simulink model "RB_KAIROS_impControl_compensation"  (R2020b)
settings: Solver=ode4  StartTime=0.0  StopTime=t_end  FixedStep=Ts  RelTol=1e-3
values from neighbouring files (symbols this model uses):
  am = 0.3    [RB_KAIROS_ImpControl_OpSpace_quat_2020b_safety_main.m]
  am_r = 0.3    [RB_KAIROS_ImpControl_OpSpace_quat_2020b_safety_main.m]
  Kc = diag(50*ones(6,1))    [RB_KAIROS_ImpControl_OpSpace_quat_2020b_safety_main.m]
  Kp = 2*[400;400;400;400;0;0;0]    [RB_KAIROS_ImpControl_OpSpace_quat_2020b_safety_main.m]
  Kv = [1000;1000;1000;[300;300;300;300;300;300;300]]    [RB_KAIROS_ImpControl_OpSpace_quat_2020b_safety_main.m]
  model_sample_time = 0.001    [RB_KAIROS_ImpControl_OpSpace_quat_2020b_safety_main.m]
  q_dot_0 = zeros(10,1)    [RB_KAIROS_ImpControl_OpSpace_quat_2020b_safety_main.m]
  T_i = K    [RB_KAIROS_ImpControl_OpSpace_quat_2020b_safety_main.m]
  tau_ext = [0 0 0 0 0 0 0 0 0 0 0]    [RB_KAIROS_ImpControl_OpSpace_quat_2020b_safety_main.m]
  v_SMU = 10    [RB_KAIROS_ImpControl_OpSpace_quat_2020b_safety_main.m]
  vm = 0.5    [RB_KAIROS_ImpControl_OpSpace_quat_2020b_safety_main.m]
  vm_r = 0.5    [RB_KAIROS_ImpControl_OpSpace_quat_2020b_safety_main.m]
undefined symbols (not defined in the file or in its folder): DiscIntNeverNeededParam, magnitude, q_0, T_f
libraries: simulink x4, utils x4, transformations_lib x3
(part 14 of 18)

== matlab function RB_KAIROS_impControl_compensation/CONTROLLER /Kinematics and Dynamics/Dynamics - Configuration space/MATLAB Function4 ==
  data: qv input; M output; qa input
function M = get_M(qv,qa)
%GET_M
%    M = GET_M(qv,qa)

%    This function was generated by the Symbolic Math Toolbox version 8.6.
%    14-Feb-2023 10:04:23

phi = qv(3);
q1 = qa(1);
q2 = qa(2);
q3 = qa(3);
q4 = qa(4);
q5 = qa(5);
q6 = qa(6);
q7 = qa(7);
t2 = cos(phi);
t3 = cos(q1);
t4 = cos(q2);
t5 = cos(q3);
t6 = cos(q4);
t7 = cos(q5);
t8 = cos(q6);
t9 = cos(q7);
t10 = sin(phi);
t11 = sin(q1);
t12 = sin(q2);
t13 = sin(q3);
t14 = sin(q4);
t15 = sin(q5);
t16 = sin(q6);
t17 = sin(q7);
t18 = t4.^2;
t19 = t12.^2;
t20 = t4.*t6;
t21 = t5.*t7;
t22 = t6.*t8;
t23 = t7.*t9;
t24 = t4.*t14;
t25 = t5.*t15;
t26 = t6.*t16;
t27 = t7.*t17;
t28 = -t10;
t29 = t12.*t13.*t15;
t30 = t13.*t14.*t16;
t31 = t14.*t15.*t17;
t32 = t5.*t6.*t12;
t33 = t6.*t7.*t13;
t34 = t7.*t8.*t14;
t35 = t8.*t9.*t15;
t36 = t5.*t12.*t14;
t37 = t7.*t12.*t13;
t38 = t6.*t13.*t15;
t39 = t8.*t13.*t14;
t40 = t7.*t14.*t16;
t41 = t9.*t14.*t15;
t42 = t8.*t15.*t17;
t44 = t7.*(1.1e+1./1.25e+2);
t45 = t4.*(3.3e+1./4.0e+2);
t46 = t5.*(3.3e+1./4.0e+2);
t47 = t6.*(3.3e+1./4.0e+2);
t48 = t7.*(3.3e+1./4.0e+2);
t49 = t8.*(3.3e+1./4.0e+2);
t50 = t14.*(4.8e+1./1.25e+2);
t51 = t15.*(4.8e+1./1.25e+2);
t52 = t15.*(3.3e+1./4.0e+2);
t53 = t16.*(3.3e+1./4.0e+2);
t63 = t13.*(7.9e+1./2.5e+2);
t67 = t8.*t9.*(1.1e+1./1.25e+2);
t69 = t7.*t8.*(4.8e+1./1.25e+2);
t72 = t8.*t17.*(1.1e+1./1.25e+2);
t74 = t6.*t13.*(4.8e+1./1.25e+2);
t76 = t7.*t16.*(4.8e+1./1.25e+2);
t79 = t14.*t15.*(1.1e+1./1.25e+2);
t81 = t12.*t13.*(3.3e+1./4.0e+2);
t82 = t13.*t14.*(3.3e+1./4.0e+2);
t83 = t5.*t6.*(7.9e+1./2.5e+2);
t84 = t5.*t6.*(-3.3e+1./4.0e+2);
t85 = t5.*t12.*(7.9e+1./2.5e+2);
t86 = t5.*t14.*(7.9e+1./2.5e+2);
t88 = t5.*t14.*(-3.3e+1./4.0e+2);
t93 = t4.*3.925e-3;
t94 = t12.*2.872e-2;
t95 = t12.*3.925e-3;
t96 = t15.*t16.*t17.*(1.1e+1./1.25e+2);
t100 = t13.*t15.*(-7.9e+1./2.5e+2);
t101 = t6.*1.9552e-2;
t102 = t5.*1.0442e-1;
t105 = t14.*1.0442e-1;
t115 = t9.*t15.*t16.*(1.1e+1./1.25e+2);
t121 = t12.*t13.*t14.*(-3.3e+1./4.0e+2);
t122 = t4.*1.083e-2;
t123 = t4.*2.811e-2;
t124 = t5.*5.317e-2;
t125 = t6.*5.317e-2;
t132 = t6.*t12.*t13.*(-3.3e+1./4.0e+2);
t134 = t12.*t13.*t14.*(-7.9e+1./2.5e+2);
t136 = t6.*t13.*1.0442e-1;
t137 = t13.*t14.*1.9552e-2;
t138 = t12.*t13.*1.0442e-1;
t144 = t6.*t12.*t13.*(-7.9e+1./2.5e+2);
t147 = t12.*t13.*5.317e-2;
t148 = t13.*t14.*5.317e-2;
t213 = t13.*3.7242e-2;
t214 = t7.*2.9474e-2;
t223 = t14.*t15.*2.9474e-2;
t224 = t17.*1.2516e-2;
t225 = t5.*t12.*3.7242e-2;
t229 = t8.*4.815e-3;
t230 = t15.*3.5549e-2;
t231 = t5.*1.01140545e-1;
t232 = t7.*1.01140545e-1;
t233 = t15.*1.01140545e-1;
t240 = t15.*4.1065e-2;
t241 = t12.*7.962e-3;
t242 = t8.*4.354e-3;
t243 = t4.*1.2805e-2;
t244 = t5.*1.2805e-2;
t245 = t5.*2.8323e-2;
t246 = t6.*8.626999999999999e-3;
t247 = t7.*5.433e-3;
t250 = t14.*2.5853e-2;
t251 = t4.*2.7518e-2;
t252 = t5.*2.7518e-2;
t254 = t5.*3.6155e-2;
t255 = t7.*6.0149e-2;
t256 = t8.*6.0149e-2;
t257 = t4.*3.9252e-2;
t258 = t4.*1.1396e-2;
t259 = t13.*3.9252e-2;
t262 = t13.*1.1396e-2;
t263 = t5.*8.640999999999999e-3;
t264 = t6.*8.640999999999999e-3;
t266 = t9.*t16.*1.2516e-2;
t267 = t6.*4.1065e-2;
t268 = t15.*6.3995712e-1;
t269 = t8.*1.196e-3;
t271 = t17.*4.28e-4;
t272 = t6.*7.796e-3;
t274 = t8.*1.0517e-2;
t275 = t9.*1.0517e-2;
t276 = t7.*2.117e-3;
t277 = t17.*1.196e-3;
t278 = t14.*7.796e-3;
t279 = t15.*2.117e-3;
t280 = t6.*4.037e-3;
t281 = t7.*6.4725936e-2;
t282 = t4.*3.495e-3;
t283 = t7.*t16.*2.82440448e-1;
t284 = t9.*t15.*2.82440448e-1;
t285 = t15.*4.037e-3;
t288 = t12.*3.495e-3;
t289 = t5.*t14.*3.87398936e-1;
t290 = t7.*t13.*3.87398936e-1;
t291 = t15.*t17.*2.82440448e-1;
t292 = t7.*1.158e-3;
t294 = t13.*t15.*3.87398936e-1;
t295 = t16.*1.158e-3;
t296 = t5.*1.332e-3;
t298 = t9.*1.0027e-2;
t300 = t14.*1.332e-3;
t302 = t7.*t14.*3.5549e-2;
t304 = t15.*t16.*4.815e-3;
t305 = t12.*t13.*1.01140545e-1;
t306 = t7.*t14.*3.8437e-2;
t307 = t14.*t15.*3.8437e-2;
t308 = t6.*1.1953e-2;
t309 = t7.*1.1953e-2;
t310 = t16.*1.964e-3;
t311 = t4.*3.141e-3;
t312 = t8.*4.252e-3;
t314 = t5.*4.761e-3;
t315 = t17.*4.252e-3;
t318 = t13.*4.761e-3;
t319 = t7.*1.4117e-2;
t321 = t16.*1.4117e-2;
t322 = t9.*4.28e-4;
t326 = t8.*6.0680565e-2;
t327 = t7.*3.41e-4;
t328 = t8.*3.41e-4;
t331 = t15.*t16.*4.354e-3;
t332 = t12.*t13.*1.2805e-2;
t336 = t6.*2.29e-4;
t337 = t7.*2.29e-4;
t339 = t12.*t13.*2.8323e-2;
t342 = t9.*t16.*6.1597e-2;
t345 = t13.*t14.*8.626999999999999e-3;
t346 = t16.*t17.*6.1597e-2;
t348 = t14.*t15.*5.433e-3;
t350 = t5.*t6.*(-1.01140545e-1);
t352 = t6.*t13.*2.5853e-2;
t354 = t6.*t13.*2.7454e-2;
t355 = t13.*t14.*2.7454e-2;
t360 = t8.*7.41e-4;
t361 = t9.*7.41e-4;
t362 = t12.*t13.*2.7518e-2;
t364 = t12.*t13.*3.6155e-2;
t365 = t5.*t12.*3.9252e-2;
t366 = t14.*t15.*6.0149e-2;
t367 = t15.*t16.*6.0149e-2;
t368 = t5.*t12.*1.1396e-2;
t372 = t7.*t8.*6.3995712e-1;
t375 = t7.*t16.*6.3995712e-1;
t377 = t7.*t14.*4.1065e-2;
t378 = t12.*t13.*8.640999999999999e-3;
t379 = t13.*t14.*8.640999999999999e-3;
t383 = t13.*t14.*4.1065e-2;
t384 = t15.*t16.*1.0517e-2;
t385 = t16.*t17.*1.0517e-2;
t386 = t16.*1.09e-4;
t390 = t7.*t14.*4.037e-3;
t391 = t8.*t17.*6.4725936e-2;
t393 = t13.*t14.*4.037e-3;
t394 = t14.*t15.*6.4725936e-2;
t396 = t8.*t15.*1.158e-3;
t398 = t12.*t13.*t14.*3.87398936e-1;
t399 = t14.*t15.*1.158e-3;
t401 = t7.*1.374907875e-1;
t402 = t8.*1.374907875e-1;
t404 = t6.*t13.*1.332e-3;
t409 = t16.*1.374907875e-1;
t410 = t12.*t13.*1.332e-3;
t413 = t16.*t17.*1.0027e-2;
t419 = t13.*1.13377482;
t424 = t8.*t15.*1.964e-3;
t428 = t9.*t16.*4.252e-3;
t429 = t13.*t14.*1.1953e-2;
t430 = t14.*t15.*1.1953e-2;
t433 = t15.*t16.*4.252e-3;
t436 = t8.*t15.*1.4117e-2;
t439 = t14.*t15.*1.4117e-2;
t448 = t4.*2.960013375e-1;
t450 = t9.*t16.*1.196e-3;
t456 = t8.*1.09e-4;
t459 = t15.*t16.*1.196e-3;
t463 = t8.*t9.*6.4725936e-2;
t465 = t14.*t15.*3.41e-4;
t466 = t15.*t16.*3.41e-4;
t474 = t13.*t14.*2.29e-4;
t475 = t14.*t15.*2.29e-4;
t488 = t6.*t12.*t13.*(-1.01140545e-1);
t496 = t15.*t16.*7.41e-4;
t497 = t16.*t17.*7.41e-4;
t512 = t6.*t13.*(-7.796e-3);
t513 = t8.*t15.*(-1.0517e-2);
t515 = t13.*t14.*(-7.796e-3);
t529 = t5.*t6.*1.13377482;
t532 = t5.*t12.*1.13377482;
t533 = t5.*t14.*1.13377482;
t543 = t5.*t12.*2.49498e-1;
t548 = t12.*t13.*2.49498e-1;
t555 = t5.*t6.*2.960013375e-1;
t565 = t5.*t14.*2.960013375e-1;
t589 = t9.*t15.*t16.*6.4725936e-2;
t593 = t15.*t16.*t17.*6.4725936e-2;
t608 = t7.*t13.*5.2663138e-1;
t617 = t12.*1.857971472e-2;
t623 = t8.*t15.*(-1.09e-4);
t624 = t15.*t16.*(-1.09e-4);
t629 = t5.*1.9076837715e-1;
t630 = t6.*1.9076837715e-1;
t634 = t6.*t12.*t13.*2.960013375e-1;
t637 = t12.*t13.*t14.*2.960013375e-1;
t643 = t5.*3.746479959e-1;
t644 = t14.*3.746479959e-1;
t651 = t12.*t13.*1.9076837715e-1;
t652 = t13.*t14.*1.9076837715e-1;
t655 = t6.*t13.*3.746479959e-1;
t656 = t12.*t13.*3.746479959e-1;
t694 = t2.*1.224646799147353e-16;
t700 = t10.*1.224646799147353e-16;
t718 = t5.*t6.*1.02650375589525e-1;
t722 = t5.*t14.*9.119126684115e-2;
t734 = t12.*t13.*t14.*3.090845966175e-2;
t749 = t6.*t12.*t13.*1.5738391114875e-2;
t763 = t6.*t12.*t13.*1.02650375589525e-1;
t765 = t12.*t13.*t14.*9.119126684115e-2;
t772 = t5.*7.75868983449435e-2;
t789 = t12.*t13.*7.75868983449435e-2;
t870 = t4.*8.8844724872e-2;
t871 = t5.*8.8844724872e-2;
t872 = t4.*1.26729164208e-1;
t873 = t13.*1.26729164208e-1;
t874 = t6.*5.034347249e-2;
t875 = t15.*5.034347249e-2;
t876 = t7.*t14.*4.7121686402e-2;
t877 = t14.*t15.*4.7121686402e-2;
t879 = t6.*1.4653732538e-2;
t880 = t7.*1.4653732538e-2;
t887 = t7.*2.3526756935e-2;
t890 = t16.*2.3526756935e-2;
t892 = t8.*3.127439544e-3;
t893 = t17.*3.127439544e-3;
t894 = t8.*7.735484874e-3;
t895 = t9.*7.735484874e-3;
t898 = t7.*1.00241616695e-1;
t899 = t8.*1.00241616695e-1;
t900 = t12.*t13.*8.8844724872e-2;
t901 = t12.*2.26100637e-3;
t902 = t5.*t12.*1.26729164208e-1;
t905 = t6.*t13.*9.850206933e-2;
t906 = t13.*t14.*9.850206933e-2;
t912 = t7.*t14.*5.034347249e-2;
t914 = t7.*1.208932934385e-3;
t916 = t13.*t14.*5.034347249e-2;
t920 = t9.*t16.*4.5305948634e-2;
t921 = t4.*2.031994566e-3;
t922 = t15.*4.153336480425e-3;
t923 = t16.*t17.*4.5305948634e-2;
t924 = t4.*2.26100637e-3;
t927 = t13.*t15.*1.590853730684e-2;
t929 = t13.*t14.*1.4653732538e-2;
t930 = t14.*t15.*1.4653732538e-2;
t934 = t9.*t15.*2.970426191616e-3;
t937 = t8.*t15.*2.3526756935e-2;
t940 = t8.*t15.*1.7527158935e-2;
t941 = t14.*t15.*2.3526756935e-2;
t943 = t9.*t16.*3.127439544e-3;
t946 = t15.*t16.*1.7527158935e-2;
t947 = t15.*t16.*3.127439544e-3;
t951 = t15.*t16.*7.735484874e-3;
t952 = t16.*t17.*7.735484874e-3;
t957 = t8.*8.2699333773375e-3;
t958 = t14.*t15.*1.00241616695e-1;
t959 = t15.*t16.*1.00241616695e-1;
t963 = t7.*t16.*3.849278081088e-2;
t965 = t3.*2.75e-1;
t966 = t8.*t9.*6.80722668912e-4;
t967 = t11.*2.75e-1;
t972 = t3.*1.55e-1;
t974 = t11.*1.55e-1;
t975 = t7.*t13.*4.630579482008e-3;
t976 = t15.*t17.*1.200936784896e-3;
t1015 = t5.*t12.*8.055302407919999e-1;
t1017 = t12.*t13.*8.055302407919999e-1;
t1022 = t7.*t8.*9.03427466304e-3;
t1026 = t9.*t15.*t16.*6.80722668912e-4;
t1031 = t8.*t17.*2.75214679872e-4;
t1033 = t16.*1.9409574471375e-3;
t1049 = t6.*1.644586079438601e-3;
t1051 = t15.*t16.*t17.*2.75214679872e-4;
t1060 = t14.*3.9053550262761e-3;
t1065 = t13.*t14.*1.644586079438601e-3;
t1067 = t4.*7.689361029464e-4;
t1075 = t6.*t13.*3.9053550262761e-3;
t1260 = t7.*1.716784138406187e-2;
t1261 = t3.*7.704560200000002e-1;
t1262 = t11.*7.704560200000002e-1;
t1266 = t16.*1.037589172186849e-4;
t1267 = t5.*4.442367301156758e-2;
t1268 = t17.*1.672482661783778e-3;
t1270 = t9.*5.48359106408232e-4;
t1271 = t3.*1.3669381;
t1272 = t14.*t15.*2.16405205209813e-3;
t1273 = t11.*1.3669381;
t1275 = t15.*1.026787777028894e-3;
t1276 = t11.*1.0027353e-1;
t1277 = t7.*t14.*4.600245517563106e-3;
t1278 = t8.*9.3569097314605e-5;
t1289 = t8.*t15.*1.037589172186849e-4;
t1292 = t3.*1.7790465e-1;
t1296 = t13.*3.356258116611425e-2;
t1300 = t9.*t16.*1.672482661783778e-3;
t1302 = t12.*t13.*4.442367301156758e-2;
t1305 = t16.*t17.*5.48359106408232e-4;
t1315 = t15.*t16.*9.3569097314605e-5;
t1316 = t8.*4.909651967360946e-3;
t1318 = t6.*1.086951076282856e-2;
t1330 = t7.*1.179456023023895e-2;
t1333 = t5.*t12.*3.356258116611425e-2;
t1348 = t15.*t16.*4.909651967360946e-3;
t1349 = t13.*t14.*1.086951076282856e-2;
t1356 = t14.*t15.*1.179456023023895e-2;
t1357 = t12.*1.026110182100817e-2;
t1366 = t4.*1.824920229252011e-2;
t1518 = t11.*1.409188914000009e-4;
t1527 = t3.*6.90020411512e-3;
t43 = -t30;
t54 = -t32;
t55 = -t35;
t56 = -t37;
t57 = -t38;
t58 = -t40;
t59 = -t41;
t60 = -t46;
t61 = -t48;
t62 = -t49;
t64 = -t52;
t65 = t21.*(1.1e+1./1.25e+2);
t66 = t22.*(1.1e+1./1.25e+2);
t68 = t21.*(4.8e+1./1.25e+2);
t70 = t20.*(3.3e+1./4.0e+2);
t71 = t6.*t46;
t73 = t24.*(4.8e+1./1.25e+2);
t75 = t25.*(4.8e+1./1.25e+2);
t77 = t9.*t51;
t78 = t14.*t46;
t80 = t17.*t51;
t87 = t7.*t63;
t89 = t12.*t63;
t90 = t15.*t63;
t91 = -t81;
t92 = -t82;
t97 = t29.*(4.8e+1./1.25e+2);
t98 = t14.*t81;
t99 = -t86;
t103 = -t94;
t104 = -t95;
t106 = t20+t36;
t107 = t25+t33;
t108 = t26+t34;
t109 = t23+t42;
t110 = t32.*(4.8e+1./1.25e+2);
t111 = t37.*(1.1e+1./1.25e+2);
t112 = t38.*(1.1e+1./1.25e+2);
t113 = t39.*(1.1e+1./1.25e+2);
t114 = t40.*(1.1e+1./1.25e+2);
t116 = t37.*(4.8e+1./1.25e+2);
t117 = t36.*(3.3e+1./4.0e+2);
t118 = t12.*t13.*t47;
t133 = t20.*1.9552e-2;
t135 = t24.*1.0442e-1;
t139 = -t124;
t145 = t20.*5.317e-2;
t156 = -t147;
t157 = -t148;
t158 = t32.*1.0442e-1;
t159 = t36.*1.9552e-2;
t165 = t36.*5.317e-2;
t166 = t47+t50;
t169 = t53+t69;
t174 = t45+t85;
t184 = t83+t88;
t219 = -t213;
t221 = t105+t125-3.3e+1./4.0e+2;
t226 = t21.*2.9474e-2;
t228 = -t224;
t248 = -t230;
t249 = -t232;
t253 = -t233;
t260 = t37.*2.9474e-2;
t261 = t38.*2.9474e-2;
t265 = t27.*1.2516e-2;
t273 = -t241;
t286 = -t243;
t297 = t22.*4.815e-3;
t299 = -t246;
t301 = t25.*3.5549e-2;
t303 = t6.*t231;
t316 = -t259;
t324 = -t271;
t325 = t22.*4.354e-3;
t329 = -t279;
t330 = -t280;
t333 = -t285;
t334 = t20.*8.626999999999999e-3;
t335 = t23.*6.1597e-2;
t338 = -t289;
t340 = t21.*5.433e-3;
t341 = t27.*6.1597e-2;
t343 = -t294;
t344 = -t295;
t347 = -t300;
t349 = t20.*2.7454e-2;
t351 = t24.*2.5853e-2;
t353 = t24.*2.7454e-2;
t356 = -t306;
t357 = t21.*6.0149e-2;
t358 = t22.*6.0149e-2;
t363 = -t307;
t369 = t20.*8.640999999999999e-3;
t370 = -t311;
t371 = t35.*1.2516e-2;
t373 = t20.*4.1065e-2;
t374 = t25.*6.3995712e-1;
t376 = t25.*4.1065e-2;
t380 = t31.*1.2516e-2;
t381 = -t318;
t382 = -t319;
t387 = t14.*t279;
t388 = -t326;
t389 = t25.*4.037e-3;
t392 = t21.*1.158e-3;
t395 = t26.*1.158e-3;
t397 = -t332;
t400 = t23.*1.0027e-2;
t403 = t24.*1.332e-3;
t406 = -t336;
t407 = t33.*3.5549e-2;
t408 = -t339;
t411 = t39.*4.815e-3;
t412 = t40.*4.815e-3;
t414 = t29.*3.5549e-2;
t415 = t6.*t305;
t416 = -t348;
t417 = t33.*3.8437e-2;
t418 = t38.*3.8437e-2;
t420 = -t355;
t421 = t20.*1.1953e-2;
t422 = t21.*1.1953e-2;
t423 = t26.*1.964e-3;
t425 = -t360;
t426 = t22.*4.252e-3;
t427 = t27.*4.252e-3;
t431 = t12.*t314;
t432 = t21.*1.4117e-2;
t434 = t12.*t318;
t435 = t26.*1.4117e-2;
t438 = t23.*4.28e-4;
t440 = t22.*1.196e-3;
t441 = t27.*4.28e-4;
t442 = t16.*t322;
t443 = t20.*7.796e-3;
t444 = -t378;
t445 = t22.*1.0517e-2;
t446 = t23.*1.0517e-2;
t447 = t21.*2.117e-3;
t449 = t27.*1.196e-3;
t451 = t16.*t271;
t452 = t24.*7.796e-3;
t453 = t13.*t272;
t454 = t26.*1.0517e-2;
t455 = t15.*t274;
t457 = t25.*2.117e-3;
t458 = t14.*t276;
t460 = t20.*4.037e-3;
t461 = t13.*t278;
t462 = t21.*6.4725936e-2;
t464 = -t385;
t467 = t20.*2.29e-4;
t468 = t21.*2.29e-4;
t470 = t35.*6.1597e-2;
t471 = t36.*8.626999999999999e-3;
t472 = t41.*6.1597e-2;
t473 = t42.*6.1597e-2;
t476 = -t398;
t477 = -t399;
t478 = -t402;
t480 = t37.*5.433e-3;
t481 = t38.*5.433e-3;
t482 = t31.*6.1597e-2;
t484 = t32.*2.5853e-2;
t485 = t32.*2.7454e-2;
t487 = t36.*2.7454e-2;
t490 = t22.*7.41e-4;
t491 = t23.*7.41e-4;
t492 = t37.*6.0149e-2;
t493 = t38.*6.0149e-2;
t494 = t39.*6.0149e-2;
t495 = t40.*6.0149e-2;
t498 = -t429;
t499 = -t430;
t500 = t33.*4.1065e-2;
t501 = t36.*8.640999999999999e-3;
t503 = t36.*4.1065e-2;
t504 = -t436;
t505 = t29.*6.3995712e-1;
t506 = t29.*4.1065e-2;
t509 = t21.*3.41e-4;
t510 = t22.*3.41e-4;
t514 = -t459;
t516 = t39.*4.354e-3;
t517 = t40.*4.354e-3;
t518 = t37.*1.158e-3;
t519 = t38.*1.158e-3;
t520 = t32.*1.332e-3;
t522 = t30.*1.158e-3;
t524 = t41.*1.0027e-2;
t525 = t42.*1.0027e-2;
t534 = t34.*1.964e-3;
t536 = t35.*4.252e-3;
t537 = t36.*1.1953e-2;
t538 = t37.*1.1953e-2;
t539 = t38.*1.1953e-2;
t544 = t30.*1.964e-3;
t545 = -t497;
t546 = t39.*4.252e-3;
t547 = t40.*4.252e-3;
t549 = t34.*1.4117e-2;
t550 = t31.*4.252e-3;
t551 = t37.*1.4117e-2;
t552 = t38.*1.4117e-2;
t553 = t35.*4.28e-4;
t554 = t30.*1.4117e-2;
t556 = t35.*1.196e-3;
t557 = t41.*4.28e-4;
t558 = t42.*4.28e-4;
t559 = t32.*7.796e-3;
t561 = t34.*1.0517e-2;
t562 = t22.*1.09e-4;
t564 = t33.*2.117e-3;
t566 = t39.*1.196e-3;
t567 = t40.*1.196e-3;
t568 = t31.*4.28e-4;
t569 = t36.*7.796e-3;
t571 = t39.*1.0517e-2;
t572 = t40.*1.0517e-2;
t573 = t41.*1.0517e-2;
t574 = t42.*1.0517e-2;
t575 = t26.*1.09e-4;
t576 = t15.*t456;
t577 = t37.*2.117e-3;
t578 = t38.*2.117e-3;
t579 = t31.*1.196e-3;
t580 = t33.*4.037e-3;
t583 = t30.*1.0517e-2;
t584 = t15.*t386;
t585 = t29.*2.117e-3;
t586 = t36.*4.037e-3;
t587 = t37.*6.4725936e-2;
t588 = t38.*6.4725936e-2;
t590 = t34.*1.158e-3;
t592 = t29.*4.037e-3;
t594 = t36.*2.29e-4;
t595 = t37.*2.29e-4;
t596 = t38.*2.29e-4;
t599 = t21.*3.45563e-1;
t600 = t25.*3.45563e-1;
t601 = t39.*7.41e-4;
t602 = t40.*7.41e-4;
t603 = t41.*7.41e-4;
t604 = t42.*7.41e-4;
t609 = -t548;
t614 = -t565;
t619 = t37.*3.41e-4;
t620 = t38.*3.41e-4;
t621 = t39.*3.41e-4;
t622 = t40.*3.41e-4;
t631 = t6.*t12.*t419;
t632 = t12.*t14.*t419;
t633 = t34.*1.09e-4;
t635 = t39.*1.09e-4;
t636 = t40.*1.09e-4;
t639 = t30.*1.09e-4;
t640 = -t617;
t645 = -t629;
t646 = t37.*3.45563e-1;
t647 = t29.*3.45563e-1;
t650 = -t637;
t654 = t24.*3.746479959e-1;
t657 = t20.*1.9076837715e-1;
t658 = -t651;
t659 = -t652;
t668 = t32.*3.746479959e-1;
t669 = t36.*1.9076837715e-1;
t730 = t101+t278;
t740 = -t718;
t775 = t2+t700;
t783 = -t763;
t784 = -t772;
t791 = t28+t694;
t794 = -t789;
t884 = -t873;
t896 = -t876;
t897 = -t877;
t903 = t20.*9.850206933e-2;
t904 = t24.*9.850206933e-2;
t908 = t20.*5.034347249e-2;
t909 = -t887;
t911 = t25.*5.034347249e-2;
t913 = t33.*4.7121686402e-2;
t917 = t38.*4.7121686402e-2;
t918 = t23.*4.5305948634e-2;
t919 = t27.*4.5305948634e-2;
t925 = t20.*1.4653732538e-2;
t926 = t21.*1.4653732538e-2;
t932 = t21.*2.3526756935e-2;
t933 = -t906;
t935 = t22.*1.7527158935e-2;
t936 = t26.*2.3526756935e-2;
t938 = t22.*3.127439544e-3;
t939 = t26.*1.7527158935e-2;
t942 = t27.*3.127439544e-3;
t944 = t22.*7.735484874e-3;
t945 = t23.*7.735484874e-3;
t950 = -t914;
t954 = t21.*1.00241616695e-1;
t955 = t22.*1.00241616695e-1;
t956 = t21.*4.23641577598e-1;
t961 = t25.*4.23641577598e-1;
t962 = -t921;
t964 = -t922;
t968 = t32.*9.850206933e-2;
t970 = -t929;
t971 = -t930;
t973 = t36.*9.850206933e-2;
t978 = t33.*5.034347249e-2;
t979 = -t934;
t981 = -t937;
t982 = t36.*5.034347249e-2;
t983 = -t940;
t984 = t29.*5.034347249e-2;
t985 = -t952;
t986 = t35.*4.5305948634e-2;
t987 = t41.*4.5305948634e-2;
t988 = t42.*4.5305948634e-2;
t989 = -t957;
t990 = t31.*4.5305948634e-2;
t991 = -t966;
t992 = -t967;
t994 = t34.*2.3526756935e-2;
t995 = t34.*1.7527158935e-2;
t996 = t37.*2.3526756935e-2;
t997 = t38.*2.3526756935e-2;
t998 = t35.*3.127439544e-3;
t999 = -t976;
t1000 = t39.*1.7527158935e-2;
t1001 = t40.*1.7527158935e-2;
t1002 = t30.*2.3526756935e-2;
t1003 = t39.*3.127439544e-3;
t1004 = t40.*3.127439544e-3;
t1005 = t30.*1.7527158935e-2;
t1006 = t31.*3.127439544e-3;
t1007 = t39.*7.735484874e-3;
t1008 = t40.*7.735484874e-3;
t1009 = t41.*7.735484874e-3;
t1010 = t42.*7.735484874e-3;
t1011 = t37.*1.00241616695e-1;
t1012 = t38.*1.00241616695e-1;
t1013 = t39.*1.00241616695e-1;
t1014 = t40.*1.00241616695e-1;
t1018 = t37.*4.23641577598e-1;
t1021 = t29.*4.23641577598e-1;
t1023 = t36.*1.4653732538e-2;
t1024 = t37.*1.4653732538e-2;
t1025 = t38.*1.4653732538e-2;
t1038 = -t1017;
t1040 = -t1022;
t1042 = -t1026;
t1046 = -t1031;
t1047 = -t1033;
t1053 = t244+t262;
t1055 = t250+t272;
t1056 = t256+t321;
t1057 = -t1049;
t1058 = -t1051;
t1061 = t20.*1.644586079438601e-3;
t1069 = t277+t361;
t1071 = t242+t386;
t1072 = -t1067;
t1074 = t24.*3.9053550262761e-3;
t1076 = t310+t456;
t1077 = t36.*1.644586079438601e-3;
t1079 = t362+t365;
t1091 = t251+t543;
t1092 = t32.*3.9053550262761e-3;
t1119 = t240+t309+3.3e+1./4.0e+2;
t1134 = t275+t315+1.1e+1./1.25e+2;
t1166 = t7.*(t295-t328).*(-1.0./2.0);
t1172 = t16.*t17.*(t271-t298).*(-1.0./2.0);
t1175 = t14.*t15.*(t295-t328).*(-1.0./2.0);
t1176 = (t16.*t17.*(t271-t298))./2.0;
t1184 = t72+t312+t346;
t1186 = t67+t274+t342;
t1218 = t137+t263+t512;
t1274 = -t1266;
t1283 = -t1267;
t1284 = -t1268;
t1286 = -t1270;
t1287 = -t1272;
t1288 = t26.*1.037589172186849e-4;
t1291 = -t1273;
t1293 = -t1275;
t1294 = t21.*1.716784138406187e-2;
t1295 = -t1277;
t1299 = t27.*1.672482661783778e-3;
t1303 = t23.*5.48359106408232e-4;
t1304 = t38.*2.16405205209813e-3;
t1308 = t25.*1.026787777028894e-3;
t1312 = t33.*4.600245517563106e-3;
t1313 = t22.*9.3569097314605e-5;
t1317 = -t1296;
t1320 = -t1300;
t1322 = -t1302;
t1325 = t34.*1.037589172186849e-4;
t1326 = t30.*1.037589172186849e-4;
t1331 = t37.*1.716784138406187e-2;
t1334 = t35.*1.672482661783778e-3;
t1335 = -t1316;
t1336 = t31.*1.672482661783778e-3;
t1338 = t41.*5.48359106408232e-4;
t1339 = t42.*5.48359106408232e-4;
t1341 = t29.*1.026787777028894e-3;
t1344 = t39.*9.3569097314605e-5;
t1345 = t40.*9.3569097314605e-5;
t1346 = t22.*4.909651967360946e-3;
t1347 = t20.*1.086951076282856e-2;
t1355 = t21.*1.179456023023895e-2;
t1362 = -t1348;
t1363 = -t1349;
t1367 = -t1357;
t1369 = t39.*4.909651967360946e-3;
t1370 = t40.*4.909651967360946e-3;
t1371 = t36.*1.086951076282856e-2;
t1375 = t37.*1.179456023023895e-2;
t1376 = t38.*1.179456023023895e-2;
t1425 = t245+t379+t404;
t1431 = t296+t352+t515;
t1434 = t247+t396+t466;
t1440 = t292+t424+t624;
t1441 = t327+t331+t623;
t1483 = t630+t644-2.960013375e-1;
t1524 = t890+t899;
t1531 = t900+t902;
t1533 = t870+t1015;
t1539 = t965+t974;
t1553 = -t4.*(t967-t972);
t1554 = -t12.*(t967-t972);
t1573 = t4.*t5.*(t967-t972);
t1574 = t6.*t12.*(t967-t972);
t1575 = t12.*t14.*(t967-t972);
t1636 = t875+t880+1.01140545e-1;
t1649 = t893+t895+6.4725936e-2;
t1657 = t463+t894+t920;
t1658 = t391+t892+t923;
t1660 = t12.*(t967-t972).*(-3.228604);
t1664 = t12.*(t967-t972).*(-6.46926e-1);
t1666 = t4.*(t967-t972).*(-6.46926e-1);
t1667 = t4.*t13.*(t967-t972).*(-3.587895);
t1674 = t4.*t13.*(t967-t972).*(-3.228604);
t1692 = t4.*(t967-t972).*(-1.857971472e-2);
t1695 = t4.*(t967-t972).*1.857971472e-2;
t1766 = t12.*(t967-t972).*(-2.031994566e-3);
t1767 = -t13.*t870.*(t967-t972);
t1769 = -t5.*t872.*(t967-t972);
t1772 = t12.*(t967-t972).*2.031994566e-3;
t1830 = t1262+t1271+1.92614005e-2;
t119 = -t97;
t120 = t14.*t89;
t126 = -t110;
t127 = -t111;
t128 = -t112;
t129 = -t114;
t130 = -t116;
t131 = t6.*t89;
t140 = t24+t54;
t141 = t21+t57;
t142 = t22+t58;
t143 = t27+t55;
t146 = -t135;
t149 = t8.*t106;
t150 = t8.*t107;
t151 = t9.*t108;
t152 = t16.*t106;
t153 = t16.*t107;
t154 = t17.*t108;
t155 = -t145;
t167 = -t165;
t170 = t7.*t166;
t171 = t15.*t166;
t180 = t74+t92;
t182 = t9.*t169;
t183 = t17.*t169;
t185 = t7.*t174;
t186 = t15.*t174;
t197 = t7.*t184;
t198 = t15.*t184;
t199 = t104+t123;
t204 = t98+t144;
t217 = t60+t71+t86;
t236 = -t226;
t320 = -t265;
t405 = -t335;
t469 = -t392;
t479 = -t403;
t483 = -t412;
t486 = -t414;
t489 = -t417;
t502 = -t432;
t507 = -t441;
t508 = -t445;
t511 = -t447;
t521 = -t468;
t523 = -t470;
t526 = -t472;
t527 = -t473;
t528 = -t481;
t530 = -t484;
t531 = -t485;
t535 = -t490;
t540 = -t492;
t541 = -t493;
t542 = -t495;
t563 = -t505;
t581 = -t510;
t582 = t63+t136+t157;
t591 = -t517;
t597 = -t522;
t598 = -t524;
t605 = -t536;
t606 = -t539;
t607 = -t547;
t610 = -t551;
t611 = -t556;
t612 = -t557;
t613 = -t559;
t615 = -t566;
t616 = -t567;
t618 = -t572;
t625 = -t585;
t626 = -t587;
t627 = -t588;
t628 = -t592;
t641 = -t619;
t642 = -t620;
t649 = -t636;
t653 = -t646;
t662 = -t654;
t663 = -t657;
t674 = -t669;
t706 = t93+t273;
t721 = t103+t311;
t797 = t3.*t775;
t798 = t11.*t775;
t806 = t3.*t791;
t807 = t11.*t791;
t812 = (t13.*t14.*t730)./2.0;
t885 = (t106.*t730)./2.0;
t949 = -t913;
t960 = -t918;
t977 = -t932;
t980 = -t935;
t993 = -t968;
t1016 = -t986;
t1019 = -t987;
t1020 = -t988;
t1027 = t219+t314;
t1028 = -t996;
t1029 = -t998;
t1030 = -t1004;
t1032 = -t1008;
t1034 = t214+t329;
t1035 = -t1011;
t1036 = -t1012;
t1037 = -t1014;
t1039 = -t1018;
t1041 = -t1025;
t1052 = t228+t322;
t1054 = t248+t276;
t1059 = t252+t316;
t1063 = t71+t86+t139+t354;
t1064 = t102+t184+t420;
t1066 = t264+t347;
t1068 = t254+t381;
t1070 = -t1061;
t1073 = t298+t324;
t1080 = t328+t344;
t1081 = t333+t337;
t1082 = -t1077;
t1105 = -t1092;
t1106 = (t4.*t1053)./2.0;
t1107 = t257+t609;
t1109 = t377+t499;
t1116 = t428+t464;
t1150 = (t6.*t13.*t1055)./2.0;
t1152 = (t8.*t1069)./2.0;
t1168 = (t15.*t16.*t1069)./2.0;
t1170 = (t15.*t16.*t1071)./2.0;
t1174 = (t8.*t15.*t1076)./2.0;
t1189 = t51+t367+t504;
t1219 = t122+t368+t397;
t1235 = t109.*(t271-t298).*(-1.0./2.0);
t1247 = (t108.*t1076)./2.0;
t1263 = t62+t76+t255+t513;
t1264 = (t6.*t1218)./2.0;
t1265 = t169+t382+t384;
t1307 = -t1288;
t1311 = -t1294;
t1319 = -t1299;
t1323 = -t1303;
t1324 = -t1304;
t1332 = -t1312;
t1340 = -t1325;
t1342 = -t1331;
t1350 = -t1336;
t1351 = -t1338;
t1352 = -t1339;
t1359 = -t1344;
t1360 = -t1345;
t1361 = -t1346;
t1365 = -t1355;
t1382 = -t1375;
t1384 = (t106.*t1218)./2.0;
t1400 = t225+t258+t434;
t1403 = t640+t921;
t1418 = t266+t269+t451;
t1419 = t223+t406+t458;
t1428 = t286+t364+t431;
t1429 = t302+t330+t387;
t1432 = t229+t450+t545;
t1438 = t299+t390+t475;
t1439 = t413+t425+t442;
t1466 = (t14.*t1431)./2.0;
t1469 = (t12.*t13.*t1425)./2.0;
t1482 = (t14.*t15.*t1434)./2.0;
t1495 = (t16.*t1440)./2.0;
t1498 = (t8.*t1441)./2.0;
t1513 = t419+t655+t659;
t1520 = t871+t884;
t1529 = (t108.*t1440)./2.0;
t1535 = t912+t971;
t1536 = t872+t1038;
t1537 = t943+t985;
t1540 = t972+t992;
t1549 = t5.*t1539;
t1550 = t13.*t1539;
t1560 = t5.*t1553;
t1561 = t13.*t1553;
t1562 = t6.*t1554;
t1563 = t14.*t1554;
t1565 = t13.*t1091.*4.02765120396e-1;
t1568 = t1539+3.875e-3;
t1596 = t9.*t1184.*2.2652974317e-2;
t1598 = t17.*t1186.*2.2652974317e-2;
t1662 = t268+t959+t981;
t1665 = t13.*t1533.*1.24749e-1;
t1668 = t1574.*(-3.587895);
t1669 = t1575.*(-3.587895);
t1670 = t1574.*(-1.225946);
t1673 = t1573.*(-3.228604);
t1676 = t1575.*3.587895;
t1677 = t1574.*1.225946;
t1685 = t282+t1553;
t1688 = t288+t1554;
t1705 = t644.*t1554;
t1706 = t630.*t1554;
t1721 = t94+t370+t1539;
t1727 = t533+t555+t645+t905;
t1728 = t529+t614+t643+t933;
t1734 = t1284+t1286;
t1756 = t873.*t1539;
t1760 = t871.*t1539;
t1775 = t9.*t1658.*3.07985e-2;
t1776 = t17.*t1657.*3.07985e-2;
t1784 = t372+t409+t909+t946;
t1789 = t375+t478+t898+t983;
t1794 = t1079+t1554;
t1853 = t924+t1666;
t1854 = t901+t1664;
t1866 = t1649.*(t385-t428).*(-1.0./2.0);
t1886 = t1261+t1291+1.0343993404e-2;
t1906 = t631+t650+t656+t903+t973;
t2010 = t617+t962+t1276+t1292;
t2014 = t1531+t1660;
t2309 = t991+t1046+t1305+t1320+t1335;
t160 = t7.*t140;
t161 = -t149;
t162 = t9.*t141;
t163 = t15.*t140;
t164 = t17.*t141;
t172 = t149.*(1.1e+1./1.25e+2);
t173 = t153.*(1.1e+1./1.25e+2);
t176 = t39+t153;
t177 = t31+t151;
t178 = -t170;
t179 = -t171;
t188 = t43+t150;
t189 = t59+t154;
t190 = t66+t129;
t191 = -t183;
t192 = t7.*t180;
t193 = -t185;
t194 = t15.*t180;
t195 = -t186;
t201 = -t9.*(t30-t150);
t203 = -t17.*(t30-t150);
t208 = t4.*t199;
t211 = -t7.*(t131+t14.*t91);
t212 = -t15.*(t131+t14.*t91);
t216 = t15.*(t131+t14.*t91);
t237 = t8.*t217;
t239 = t16.*t217;
t359 = t91+t118+t120;
t664 = t151.*1.2516e-2;
t671 = t70+t73+t117+t126;
t673 = t149.*4.815e-3;
t675 = t153.*4.815e-3;
t676 = t149.*6.0149e-2;
t677 = t153.*6.0149e-2;
t680 = t149.*4.354e-3;
t681 = t153.*4.354e-3;
t682 = t151.*6.1597e-2;
t683 = t154.*6.1597e-2;
t685 = t150.*1.964e-3;
t687 = t152.*1.964e-3;
t688 = t149.*4.252e-3;
t689 = t151.*4.252e-3;
t690 = t153.*4.252e-3;
t691 = t150.*1.4117e-2;
t692 = t152.*1.4117e-2;
t693 = t151.*4.28e-4;
t695 = t149.*1.196e-3;
t696 = t151.*1.196e-3;
t697 = t154.*4.28e-4;
t698 = t149.*1.0517e-2;
t699 = t150.*1.0517e-2;
t701 = t153.*1.196e-3;
t703 = t152.*1.0517e-2;
t704 = t153.*1.0517e-2;
t705 = t154.*1.0517e-2;
t707 = t150.*1.158e-3;
t708 = t152.*1.158e-3;
t709 = t154.*1.0027e-2;
t711 = t153.*7.41e-4;
t712 = t154.*7.41e-4;
t725 = t149.*3.41e-4;
t728 = t153.*3.41e-4;
t737 = t149.*7.41e-4;
t743 = t149.*1.09e-4;
t744 = t150.*1.09e-4;
t746 = t152.*1.09e-4;
t747 = t153.*1.09e-4;
t774 = t170.*1.666555;
t779 = t170.*1.225946;
t780 = t12.*t706;
t781 = t171.*1.225946;
t787 = t182.*7.35522e-1;
t788 = t183.*7.35522e-1;
t793 = t185.*1.666555;
t795 = t185.*1.225946;
t796 = t186.*1.225946;
t805 = -t798;
t808 = t198.*1.666555;
t809 = t197.*1.225946;
t810 = t198.*1.225946;
t814 = t9.*(t30-t150).*(-1.2516e-2);
t817 = -t812;
t822 = t9.*(t30-t150).*(-6.1597e-2);
t824 = t17.*(t30-t150).*(-6.1597e-2);
t827 = t9.*(t30-t150).*(-1.196e-3);
t828 = t17.*(t30-t150).*(-4.28e-4);
t832 = t17.*(t30-t150).*(-1.0517e-2);
t836 = t7.*(t131+t14.*t91).*(-1.225946);
t837 = t9.*(t30-t150).*6.1597e-2;
t838 = t17.*(t30-t150).*(-1.0027e-2);
t840 = t17.*(t30-t150).*6.1597e-2;
t842 = t9.*(t30-t150).*(-4.252e-3);
t846 = t9.*(t30-t150).*(-4.28e-4);
t847 = t9.*(t30-t150).*1.196e-3;
t855 = t17.*(t30-t150).*(-7.41e-4);
t856 = t9.*(t30-t150).*4.252e-3;
t1087 = t151.*4.5305948634e-2;
t1089 = t154.*4.5305948634e-2;
t1093 = t152.*1.7527158935e-2;
t1094 = t153.*1.7527158935e-2;
t1095 = t153.*3.127439544e-3;
t1096 = t149.*7.735484874e-3;
t1098 = t153.*7.735484874e-3;
t1099 = t154.*7.735484874e-3;
t1100 = t149.*1.00241616695e-1;
t1102 = t153.*1.00241616695e-1;
t1103 = (t5.*t12.*t1027)./2.0;
t1108 = (t14.*t15.*t1034)./2.0;
t1110 = t150.*2.3526756935e-2;
t1111 = t149.*1.7527158935e-2;
t1112 = t150.*1.7527158935e-2;
t1113 = t152.*2.3526756935e-2;
t1114 = t149.*3.127439544e-3;
t1115 = t151.*3.127439544e-3;
t1124 = -t1106;
t1142 = (t9.*t16.*t1052)./2.0;
t1147 = (t5.*t1066)./2.0;
t1149 = (t7.*t14.*t1054)./2.0;
t1161 = (t6.*t1081)./2.0;
t1162 = (t12.*t13.*t1068)./2.0;
t1164 = (t12.*t13.*t1066)./2.0;
t1169 = t171.*5.034347249e-2;
t1173 = t170.*1.4653732538e-2;
t1177 = (t13.*t14.*t1081)./2.0;
t1178 = -t1174;
t1179 = t182.*3.127439544e-3;
t1180 = t797.*4.970684;
t1181 = t186.*5.034347249e-2;
t1182 = t183.*7.735484874e-3;
t1183 = t798.*4.970684;
t1185 = t146+t155+t158+t167+t174;
t1187 = t797.*6.46926e-1;
t1188 = t798.*6.46926e-1;
t1193 = t185.*1.4653732538e-2;
t1197 = t197.*5.034347249e-2;
t1198 = (t141.*t1034)./2.0;
t1199 = t806.*4.970684;
t1200 = t807.*4.970684;
t1202 = t17.*(t30-t150).*(-4.5305948634e-2);
t1205 = t806.*6.46926e-1;
t1206 = t807.*6.46926e-1;
t1207 = t198.*1.4653732538e-2;
t1208 = (t107.*t1054)./2.0;
t1211 = t9.*(t30-t150).*(-4.5305948634e-2);
t1212 = t17.*(t30-t150).*4.5305948634e-2;
t1215 = t797.*1.92614005e-2;
t1216 = (t143.*t1052)./2.0;
t1217 = t798.*1.92614005e-2;
t1222 = t9.*(t30-t150).*(-3.127439544e-3);
t1226 = t17.*(t30-t150).*(-7.735484874e-3);
t1229 = t9.*(t30-t150).*4.5305948634e-2;
t1236 = t9.*(t30-t150).*3.127439544e-3;
t1239 = (t140.*t1055)./2.0;
t1243 = t7.*(t131+t14.*t91).*(-5.034347249e-2);
t1244 = (t106.*t1081)./2.0;
t1248 = (t142.*t1071)./2.0;
t1249 = t806.*1.92614005e-2;
t1251 = t807.*1.92614005e-2;
t1252 = t4.*t1219;
t1254 = (t142.*t1069)./2.0;
t1255 = t141.*(t295-t328).*(-1.0./2.0);
t1259 = (t141.*(t295-t328))./2.0;
t1269 = -t1264;
t1372 = ((t41-t154).*(t271-t298))./2.0;
t1379 = t64+t171+t267+t363;
t1381 = t1076.*(t30-t150).*(-1.0./2.0);
t1383 = t61+t170+t308+t356;
t1386 = -t1384;
t1387 = t150.*1.037589172186849e-4;
t1388 = t152.*1.037589172186849e-4;
t1393 = t154.*5.48359106408232e-4;
t1399 = t151.*1.672482661783778e-3;
t1405 = t149.*9.3569097314605e-5;
t1406 = t153.*9.3569097314605e-5;
t1420 = t149.*4.909651967360946e-3;
t1421 = t153.*4.909651967360946e-3;
t1422 = t797+t807;
t1427 = t5.*t12.*t1400;
t1430 = (t13.*t1400)./2.0;
t1442 = (t17.*t1418)./2.0;
t1443 = t797.*1.0343993404e-2;
t1445 = t798.*1.0343993404e-2;
t1450 = -t5.*(t798-t806);
t1451 = (t7.*t1419)./2.0;
t1452 = -t13.*(t798-t806);
t1453 = t12.*t13.*t1428;
t1454 = t121+t131+t138+t349+t487;
t1455 = (t5.*t1428)./2.0;
t1456 = (t15.*t1429)./2.0;
t1461 = -t6.*t12.*(t798-t806);
t1463 = -t12.*t14.*(t798-t806);
t1465 = t118+t120+t156+t353+t531;
t1470 = t806.*1.0343993404e-2;
t1472 = t807.*1.0343993404e-2;
t1474 = t9.*(t30-t150).*(-1.672482661783778e-3);
t1475 = t4.*t5.*(t798-t806);
t1476 = t17.*(t30-t150).*(-5.48359106408232e-4);
t1477 = t12.*t14.*(t798-t806);
t1485 = (t9.*t1439)./2.0;
t1486 = t9.*(t30-t150).*1.672482661783778e-3;
t1487 = (t15.*t16.*t1432)./2.0;
t1492 = (t13.*t14.*t1438)./2.0;
t1505 = -t1495;
t1514 = (t141.*t1419)./2.0;
t1515 = (t107.*t1429)./2.0;
t1516 = (t143.*t1418)./2.0;
t1519 = (t106.*t1438)./2.0;
t1521 = (t142.*t1432)./2.0;
t1522 = (t141.*t1434)./2.0;
t1525 = (t140.*t1431)./2.0;
t1526 = (t109.*t1439)./2.0;
t1532 = -t1529;
t1534 = (t142.*t1441)./2.0;
t1541 = t6.*t1064.*4.9251034665e-2;
t1542 = t14.*t1063.*4.9251034665e-2;
t1558 = -t1550;
t1567 = t1439.*(t41-t154).*(-1.0./2.0);
t1570 = -t1565;
t1571 = t5.*t1107.*4.02765120396e-1;
t1572 = t1440.*(t30-t150).*(-1.0./2.0);
t1578 = (t1440.*(t30-t150))./2.0;
t1581 = t5.*(t798-t806).*(-3.587895);
t1585 = t5.*(t798-t806).*(-3.228604);
t1588 = t13.*(t798-t806).*(-3.228604);
t1592 = t133+t159+t444+t452+t613;
t1595 = t6.*t12.*(t798-t806).*(-1.225946);
t1600 = t4.*t13.*(t798-t806).*(-3.587895);
t1601 = t6.*t12.*(t798-t806).*(-3.587895);
t1605 = -t1596;
t1621 = t4.*(t798-t806).*(-1.857971472e-2);
t1628 = t6.*t12.*(t798-t806).*(-1.9076837715e-1);
t1629 = t12.*t644.*(t798-t806);
t1630 = t12.*t630.*(t798-t806);
t1631 = t8.*t1265.*8.7635794675e-3;
t1634 = t16.*t1263.*8.7635794675e-3;
t1635 = t80+t96+t182+t405+t433+t527;
t1644 = (t221.*t1513)./2.0;
t1648 = (t582.*t1483)./2.0;
t1654 = t1550.*3.228604;
t1655 = t1549.*3.587895;
t1659 = t1549.*3.228604;
t1663 = t1540+2.081e-3;
t1672 = -t1665;
t1675 = t5.*t1536.*1.24749e-1;
t1689 = t5.*(t798-t806).*(-8.8844724872e-2);
t1691 = t13.*(t798-t806).*(-1.26729164208e-1);
t1694 = t871.*(t798-t806);
t1696 = t12.*(t798-t806).*(-2.031994566e-3);
t1697 = t4.*t13.*(t798-t806).*(-8.8844724872e-2);
t1701 = t13.*t870.*(t798-t806);
t1702 = t5.*t872.*(t798-t806);
t1707 = t18.*(t798-t806).*(-2.26100637e-3);
t1708 = t19.*(t798-t806).*(-2.26100637e-3);
t1713 = t18.*(t798-t806).*2.26100637e-3;
t1714 = t19.*(t798-t806).*2.26100637e-3;
t1722 = t44+t62+t76+t427+t446+t574+t605;
t1724 = t236+t261+t457+t474+t564;
t1725 = t46+t84+t99+t376+t422+t500+t606;
t1729 = t320+t371+t438+t514+t558;
t1730 = t301+t393+t407+t511+t578;
t1732 = t351+t410+t443+t530+t569;
t1733 = t369+t408+t479+t501+t520;
t1738 = t304+t449+t491+t604+t611;
t1742 = t345+t389+t521+t580+t596;
t1743 = t400+t496+t507+t525+t553;
t1746 = t395+t416+t581+t590+t622;
t1751 = t325+t465+t575+t591+t633;
t1757 = t423+t477+t534+t562+t649;
t1761 = t1550.*(-1.26729164208e-1);
t1780 = -t1775;
t1785 = (t1059.*t1531)./2.0;
t1786 = (t1079.*t1520)./2.0;
t1797 = (t1119.*t1535)./2.0;
t1805 = (t1134.*t1537)./2.0;
t1810 = t12.*t1059.*(t798-t806).*(-1.614302);
t1812 = (t1189.*t1524)./2.0;
t1814 = t12.*t1059.*(t798-t806).*1.614302;
t1815 = t12.*t1079.*(t798-t806).*(-1.614302);
t1817 = t12.*t1079.*(t798-t806).*1.614302;
t1822 = t14.*t1727.*1.3727e-2;
t1825 = t6.*t1728.*1.3727e-2;
t1828 = t1403.*(t798-t806).*(-1.0./2.0);
t1858 = (t1109.*t1636)./2.0;
t1859 = t4.*t1685.*1.130503185e-3;
t1860 = t12.*t1688.*1.130503185e-3;
t1864 = t8.*t1784.*5.2585e-3;
t1868 = t16.*t1789.*5.2585e-3;
t1874 = (t1056.*t1662)./2.0;
t1878 = t12.*t1520.*(t798-t806).*(-1.0./2.0);
t1881 = (t12.*t1520.*(t798-t806))./2.0;
t1882 = t12.*t1531.*(t798-t806).*(-1.0./2.0);
t1884 = (t12.*t1531.*(t798-t806))./2.0;
t1897 = t448+t532+t662+t663+t668+t674;
t1911 = t632+t634+t658+t904+t993;
t1955 = t4.*t1853.*1.7475e-3;
t1958 = t12.*t1854.*1.7475e-3;
t1987 = t89+t1550+t1573;
t1990 = (t1403.*t1721)./2.0;
t1994 = t6.*t1906.*1.3727e-2;
t2007 = t174+t1549+t1561;
t2061 = t4.*t1685.*(t798-t806).*(-3.23463e-1);
t2063 = t12.*t1688.*(t798-t806).*(-3.23463e-1);
t2065 = t4.*t1685.*(t798-t806).*3.23463e-1;
t2066 = t12.*t1688.*(t798-t806).*3.23463e-1;
t2110 = (t1064.*t1906)./2.0;
t2122 = t1830.*(t798-t806).*(-1.0./2.0);
t2123 = (t1830.*(t798-t806))./2.0;
t2128 = (t1520.*t1794)./2.0;
t2134 = (t1531.*t1794)./2.0;
t2140 = (t721.*t2010)./2.0;
t2148 = t4.*t1853.*(t798-t806).*(-1.0./2.0);
t2149 = t1091+t1549+t1561;
t2151 = t12.*t1854.*(t798-t806).*(-1.0./2.0);
t2157 = (t4.*t1853.*(t798-t806))./2.0;
t2158 = (t12.*t1854.*(t798-t806))./2.0;
t2171 = t12.*t1794.*(t798-t806).*(-1.614302);
t2174 = t12.*t1794.*(t798-t806).*1.614302;
t2200 = t1886.*(t798-t806).*(-1.0./2.0);
t2202 = (t1886.*(t798-t806))./2.0;
t2211 = t231+t338+t350+t911+t926+t978+t1041;
t2212 = (t1059.*t2014)./2.0;
t2215 = (t1079.*t2014)./2.0;
t2219 = t281+t283+t388+t942+t945+t1010+t1029;
t2278 = t2010.*(t798-t806).*(-1.0./2.0);
t2281 = (t2010.*(t798-t806))./2.0;
t2290 = t12.*t2014.*(t798-t806).*(-1.0./2.0);
t2295 = (t12.*t2014.*(t798-t806))./2.0;
t2303 = t5.*(-t1107+t1550+t1573).*(-4.02765120396e-1);
t2305 = t5.*(-t1107+t1550+t1573).*4.02765120396e-1;
t2404 = t1536.*(-t1107+t1550+t1573).*(-1.0./2.0);
t168 = -t164;
t175 = -t172;
t181 = t163.*(1.1e+1./1.25e+2);
t187 = t29+t160;
t196 = t56+t163;
t205 = t9.*t190;
t206 = t17.*t190;
t207 = -t194;
t209 = -t9.*(t37-t163);
t210 = -t17.*(t37-t163);
t215 = t48+t178;
t218 = t52+t179;
t222 = t113+t173;
t323 = -t239;
t560 = t8.*t359;
t570 = t16.*t359;
t661 = t162+t203;
t667 = t163.*2.9474e-2;
t678 = t164.*1.2516e-2;
t684 = t160.*3.8437e-2;
t686 = t163.*3.8437e-2;
t710 = t160.*3.5549e-2;
t714 = -t685;
t716 = -t688;
t717 = t163.*6.0149e-2;
t719 = -t691;
t720 = t160.*4.1065e-2;
t723 = -t698;
t724 = -t699;
t726 = -t701;
t727 = -t705;
t729 = t7.*t671;
t731 = t15.*t671;
t732 = t162.*6.1597e-2;
t733 = t164.*6.1597e-2;
t735 = t163.*5.433e-3;
t738 = -t712;
t739 = t163.*1.1953e-2;
t741 = t164.*4.252e-3;
t742 = t163.*1.4117e-2;
t745 = t162.*4.28e-4;
t748 = t164.*4.28e-4;
t750 = t162.*1.0517e-2;
t751 = -t725;
t752 = t160.*2.117e-3;
t753 = t164.*1.196e-3;
t754 = t163.*2.117e-3;
t755 = t160.*4.037e-3;
t756 = t163.*6.4725936e-2;
t757 = t163.*1.158e-3;
t758 = t162.*1.0027e-2;
t761 = -t737;
t766 = -t744;
t769 = t163.*3.41e-4;
t777 = t163.*2.29e-4;
t782 = t162.*7.41e-4;
t785 = -t774;
t790 = -t780;
t792 = -t788;
t800 = -t795;
t801 = -t796;
t802 = t192.*1.666555;
t803 = t192.*1.225946;
t804 = t194.*1.225946;
t820 = t17.*(t37-t163).*(-1.2516e-2);
t833 = t216.*(-1.666555);
t839 = t216.*(-1.225946);
t851 = t9.*(t37-t163).*(-6.1597e-2);
t852 = t216.*1.225946;
t853 = t17.*(t37-t163).*(-6.1597e-2);
t858 = t17.*(t37-t163).*(-4.28e-4);
t859 = t9.*(t37-t163).*(-1.0517e-2);
t860 = t17.*(t37-t163).*(-1.196e-3);
t861 = t9.*(t37-t163).*(-1.0027e-2);
t862 = t17.*(t37-t163).*6.1597e-2;
t863 = t17.*(t37-t163).*(-4.252e-3);
t865 = t9.*(t37-t163).*(-4.28e-4);
t867 = t298.*(t37-t163);
t868 = t9.*(t37-t163).*(-7.41e-4);
t869 = t322.*(t37-t163);
t882 = t237.*7.35522e-1;
t886 = t237.*1.666555;
t889 = t239.*1.666555;
t1062 = t75+t87+t192+t198;
t1084 = t160.*4.7121686402e-2;
t1086 = t163.*4.7121686402e-2;
t1117 = t160.*5.034347249e-2;
t1118 = -t1096;
t1120 = -t1099;
t1121 = t162.*4.5305948634e-2;
t1122 = t164.*4.5305948634e-2;
t1126 = -t1110;
t1127 = -t1111;
t1128 = -t1112;
t1129 = -t1114;
t1131 = t164.*3.127439544e-3;
t1132 = t162.*7.735484874e-3;
t1137 = t163.*1.00241616695e-1;
t1144 = t163.*1.4653732538e-2;
t1148 = t163.*2.3526756935e-2;
t1156 = -t1142;
t1158 = -t1147;
t1167 = -t1161;
t1171 = -t1164;
t1190 = -t1179;
t1191 = -t1181;
t1192 = -t1183;
t1194 = -t1188;
t1195 = t194.*5.034347249e-2;
t1196 = -t1193;
t1201 = t192.*1.4653732538e-2;
t1203 = -t1197;
t1204 = -t1198;
t1230 = t17.*(t37-t163).*(-4.5305948634e-2);
t1233 = -t1215;
t1234 = -t1216;
t1241 = t9.*(t37-t163).*(-4.5305948634e-2);
t1242 = t17.*(t37-t163).*4.5305948634e-2;
t1245 = t17.*(t37-t163).*(-3.127439544e-3);
t1246 = t9.*(t37-t163).*(-7.735484874e-3);
t1250 = -t1244;
t1253 = t216.*(-1.4653732538e-2);
t1256 = -t1249;
t1257 = -t1251;
t1258 = t216.*1.4653732538e-2;
t1281 = t239.*2.3526756935e-2;
t1285 = t237.*1.00241616695e-1;
t1310 = (t177.*t1052)./2.0;
t1343 = t1034.*(t37-t163).*(-1.0./2.0);
t1354 = (t176.*t1069)./2.0;
t1358 = (t176.*t1071)./2.0;
t1377 = -t1372;
t1385 = ((t37-t163).*(t295-t328))./2.0;
t1394 = t163.*2.16405205209813e-3;
t1395 = -t1387;
t1396 = -t1388;
t1407 = t160.*4.600245517563106e-3;
t1408 = -t1399;
t1410 = -t1406;
t1413 = t164.*1.672482661783778e-3;
t1415 = t162.*5.48359106408232e-4;
t1424 = -t1420;
t1426 = t163.*1.179456023023895e-2;
t1433 = t805+t806;
t1435 = -t1430;
t1436 = t5.*t1422;
t1437 = t13.*t1422;
t1447 = t6.*t12.*t1422;
t1448 = t12.*t14.*t1422;
t1457 = t4.*t1450;
t1459 = t4.*t1452;
t1464 = -t1456;
t1479 = -t1470;
t1491 = t1052.*(t164+t9.*(t30-t150)).*(-1.0./2.0);
t1494 = -t1485;
t1496 = t17.*(t37-t163).*(-1.672482661783778e-3);
t1497 = t9.*(t37-t163).*(-5.48359106408232e-4);
t1502 = (t1052.*(t164+t9.*(t30-t150)))./2.0;
t1507 = t1268.*(t37-t163);
t1508 = t1270.*(t37-t163);
t1517 = -t1514;
t1523 = -t1519;
t1528 = -t1522;
t1530 = -t1526;
t1538 = (t177.*t1418)./2.0;
t1548 = (t176.*t1432)./2.0;
t1555 = t1419.*(t37-t163).*(-1.0./2.0);
t1564 = (t176.*t1441)./2.0;
t1566 = t1434.*(t37-t163).*(-1.0./2.0);
t1577 = -t1571;
t1597 = t1475.*(-3.228604);
t1599 = t4.*t1588;
t1602 = t1477.*(-3.587895);
t1606 = t1475.*3.228604;
t1607 = t1477.*3.587895;
t1616 = t4.*t1422.*1.857971472e-2;
t1619 = (t6.*t1592)./2.0;
t1622 = (t13.*t14.*t1592)./2.0;
t1624 = t12.*t644.*t1422;
t1625 = t12.*t630.*t1422;
t1627 = t1477.*(-3.746479959e-1);
t1632 = t106.*t1592;
t1633 = t1418.*(t164+t9.*(t30-t150)).*(-1.0./2.0);
t1640 = t77+t115+t191+t341+t384+t523;
t1652 = t7.*t1379.*2.11820788799e-1;
t1653 = t15.*t1383.*2.11820788799e-1;
t1661 = -t1654;
t1671 = t1180+t1200;
t1679 = -t1675;
t1680 = t1187+t1206;
t1681 = t871.*t1422;
t1683 = t873.*t1422;
t1686 = t12.*t1422.*2.031994566e-3;
t1698 = t1475.*(-1.26729164208e-1);
t1699 = t18.*t1422.*2.26100637e-3;
t1700 = t19.*t1422.*2.26100637e-3;
t1709 = t87+t192+t198+t489+t498+t600;
t1712 = t6.*t1454.*4.9251034665e-2;
t1720 = t14.*t1465.*4.9251034665e-2;
t1731 = (t7.*t1724)./2.0;
t1735 = (t14.*t15.*t1724)./2.0;
t1744 = (t17.*t1729)./2.0;
t1745 = (t15.*t1730)./2.0;
t1749 = t12.*t13.*t1733;
t1750 = (t9.*t16.*t1729)./2.0;
t1752 = (t14.*t1732)./2.0;
t1753 = (t5.*t1733)./2.0;
t1755 = (t7.*t14.*t1730)./2.0;
t1762 = (t6.*t13.*t1732)./2.0;
t1763 = (t8.*t1738)./2.0;
t1764 = (t6.*t1742)./2.0;
t1765 = (t9.*t1743)./2.0;
t1768 = (t7.*t1746)./2.0;
t1771 = (t8.*t1751)./2.0;
t1774 = (t16.*t17.*t1743)./2.0;
t1778 = (t15.*t16.*t1751)./2.0;
t1779 = (t16.*t1757)./2.0;
t1781 = (t8.*t15.*t1757)./2.0;
t1783 = (t1185.*t1483)./2.0;
t1787 = t140.*t1732;
t1790 = (t106.*t1742)./2.0;
t1791 = (t142.*t1738)./2.0;
t1793 = (t141.*t1746)./2.0;
t1795 = (t1185.*t1513)./2.0;
t1796 = t253+t781+t874+t897;
t1800 = t1724.*(t37-t163).*(-1.0./2.0);
t1801 = -t1797;
t1802 = t249+t779+t879+t896;
t1803 = t12.*t1059.*t1422.*1.614302;
t1804 = (t177.*t1729)./2.0;
t1813 = t12.*t1079.*t1422.*1.614302;
t1816 = (t176.*t1738)./2.0;
t1819 = (t1403.*t1422)./2.0;
t1820 = t1743.*(t41-t154).*(-1.0./2.0);
t1821 = (t176.*t1751)./2.0;
t1824 = (t1743.*(t41-t154))./2.0;
t1827 = t9.*t1635.*2.2652974317e-2;
t1836 = t1746.*(t37-t163).*(-1.0./2.0);
t1837 = t1757.*(t30-t150).*(-1.0./2.0);
t1839 = (t1746.*(t37-t163))./2.0;
t1856 = t1729.*(t164+t9.*(t30-t150)).*(-1.0./2.0);
t1857 = (t1729.*(t164+t9.*(t30-t150)))./2.0;
t1861 = -t1858;
t1872 = (t12.*t1422.*t1520)./2.0;
t1880 = (t12.*t1422.*t1531)./2.0;
t1883 = t380+t440+t612+t616+t664+t697;
t1892 = t340+t528+t597+t621+t707+t728;
t1894 = t535+t568+t598+t602+t693+t709;
t1989 = (t221.*t1897)./2.0;
t1993 = -t1990;
t1995 = t6.*t1987;
t1996 = t14.*t1987;
t1998 = t14.*t1911.*1.3727e-2;
t2012 = (t582.*t1897)./2.0;
t2017 = t7.*t2007;
t2018 = t15.*t2007;
t2031 = (t1454.*t1728)./2.0;
t2032 = (t1465.*t1727)./2.0;
t2059 = t4.*t1422.*t1685.*3.23463e-1;
t2060 = t12.*t1422.*t1688.*3.23463e-1;
t2064 = (t1537.*t1722)./2.0;
t2067 = (t1535.*t1725)./2.0;
t2087 = t291+t593+t787+t947+t960+t1020;
t2098 = (t1635.*t1658)./2.0;
t2114 = (t1063.*t1911)./2.0;
t2117 = (t1422.*t1830)./2.0;
t2136 = (t1636.*t1725)./2.0;
t2138 = (t1649.*t1722)./2.0;
t2141 = (t4.*t1422.*t1853)./2.0;
t2143 = (t12.*t1422.*t1854)./2.0;
t2145 = -t2140;
t2164 = t1107+t1558+t1560;
t2165 = t12.*t1422.*t1794.*1.614302;
t2182 = t1185+t1549+t1561;
t2186 = t875.*t2007;
t2187 = t880.*t2007;
t2196 = (t1422.*t1886)./2.0;
t2267 = (t1422.*t2010)./2.0;
t2284 = (t12.*t1422.*t2014)./2.0;
t2301 = t13.*t2149.*4.02765120396e-1;
t2336 = (t1109.*t2211)./2.0;
t2337 = (t1119.*t2211)./2.0;
t2341 = t2219.*(t385-t428).*(-1.0./2.0);
t2342 = (t1134.*t2219)./2.0;
t2353 = t1533+t1659+t1674;
t2379 = (t1533.*t2149)./2.0;
t2421 = t5.*(-t872+t1017+t1573.*3.228604+t1654).*(-1.24749e-1);
t2423 = t5.*(-t872+t1017+t1573.*3.228604+t1654).*1.24749e-1;
t2466 = t1107.*(-t872+t1017+t1573.*3.228604+t1654).*(-1.0./2.0);
t2499 = t1655+t1667+t1897;
t200 = t8.*t187;
t202 = t16.*t187;
t227 = t16.*t218;
t234 = t9.*t215;
t235 = t17.*t215;
t238 = t8.*t218;
t287 = t9.*t222;
t293 = t17.*t222;
t638 = -t560;
t670 = t168+t201;
t672 = -t667;
t702 = -t678;
t713 = -t684;
t715 = -t686;
t736 = -t710;
t759 = -t732;
t760 = -t735;
t762 = -t739;
t764 = -t742;
t767 = -t748;
t768 = -t752;
t770 = -t754;
t771 = -t755;
t773 = -t729;
t776 = -t731;
t778 = -t757;
t786 = -t777;
t811 = -t804;
t813 = t206.*7.35522e-1;
t818 = t205.*7.35522e-1;
t910 = -t889;
t1043 = t560.*7.35522e-1;
t1044 = t560.*1.666555;
t1045 = t570.*1.666555;
t1083 = t68+t100+t197+t207;
t1088 = t9.*t1062;
t1090 = t17.*t1062;
t1101 = -t1084;
t1104 = -t1086;
t1138 = -t1121;
t1151 = t729.*1.666555;
t1154 = t729.*1.225946;
t1155 = t731.*1.225946;
t1157 = -t1144;
t1160 = -t1148;
t1213 = t206.*3.127439544e-3;
t1214 = t205.*7.735484874e-3;
t1298 = -t1281;
t1306 = -t1285;
t1329 = -t1310;
t1353 = (t187.*t1054)./2.0;
t1364 = -t1354;
t1368 = -t1358;
t1373 = t570.*2.3526756935e-2;
t1374 = t560.*1.00241616695e-1;
t1404 = -t1394;
t1411 = -t1407;
t1417 = t731.*5.034347249e-2;
t1423 = t729.*1.4653732538e-2;
t1444 = t4.*t1436;
t1446 = t4.*t1437;
t1458 = t130+t195+t211+t731;
t1462 = -t1447;
t1467 = t97+t193+t216+t729;
t1506 = t661.*(t271-t298).*(-1.0./2.0);
t1511 = (t661.*(t271-t298))./2.0;
t1544 = t893.*t1062;
t1545 = t895.*t1062;
t1551 = (t187.*t1429)./2.0;
t1552 = -t1548;
t1569 = -t1564;
t1576 = t1436.*3.587895;
t1579 = t1436.*3.228604;
t1580 = t1437.*3.228604;
t1582 = t1447.*1.225946;
t1587 = t1447.*3.587895;
t1589 = t1448.*3.587895;
t1620 = -t1616;
t1626 = -t1622;
t1643 = (t661.*t1439)./2.0;
t1656 = -t1653;
t1678 = t1192+t1199;
t1682 = t1194+t1205;
t1684 = t1436.*(-8.8844724872e-2);
t1687 = t870.*t1437;
t1690 = t872.*t1436;
t1693 = -t1686;
t1711 = t100+t197+t207+t383+t418+t599;
t1723 = t215+t358+t435+t542+t549;
t1747 = -t1744;
t1748 = -t1745;
t1754 = -t1750;
t1758 = -t1749;
t1759 = -t1753;
t1770 = -t1764;
t1773 = -t1768;
t1777 = -t1774;
t1782 = -t1781;
t1788 = -t1783;
t1792 = -t1790;
t1798 = -t1795;
t1808 = -t1804;
t1811 = (t187.*t1730)./2.0;
t1818 = -t1816;
t1826 = -t1821;
t1829 = -t1827;
t1833 = t17.*t1640.*2.2652974317e-2;
t1835 = (t721.*t1680)./2.0;
t1840 = t1436+t1459;
t1843 = t1437+t1475;
t1863 = (t661.*t1743)./2.0;
t1869 = t15.*t1709.*2.11820788799e-1;
t1879 = t494+t554+t677+t719+t1062;
t1887 = t297+t483+t579+t603+t696+t738;
t1888 = t7.*t1796.*1.727815e-1;
t1889 = t15.*t1802.*1.727815e-1;
t1891 = (t17.*t1883)./2.0;
t1895 = (t9.*t16.*t1883)./2.0;
t1898 = t469+t519+t544+t635+t714+t747;
t1900 = t509+t516+t639+t642+t681+t766;
t1904 = (t7.*t1892)./2.0;
t1912 = (t14.*t15.*t1892)./2.0;
t1913 = (t9.*t1894)./2.0;
t1920 = (t16.*t17.*t1894)./2.0;
t1944 = (t143.*t1883)./2.0;
t1954 = (t109.*t1894)./2.0;
t1980 = t1892.*(t37-t163).*(-1.0./2.0);
t1981 = (t1892.*(t37-t163))./2.0;
t1991 = -t1989;
t2000 = -t1995;
t2001 = -t1996;
t2006 = t1883.*(t164+t9.*(t30-t150)).*(-1.0./2.0);
t2015 = -t2012;
t2022 = -t2017;
t2023 = -t2018;
t2026 = (t661.*t1894)./2.0;
t2029 = t411+t675+t753+t782+t847+t855;
t2034 = t17.*(t566+t678+t701-t745+t9.*(t30-t150).*1.2516e-2+t271.*(t30-t150)).*(-1.0./2.0);
t2037 = t9.*t16.*(t566+t678+t701-t745+t9.*(t30-t150).*1.2516e-2+t271.*(t30-t150)).*(-1.0./2.0);
t2049 = (t1568.*t1671)./2.0;
t2062 = t143.*(t566+t678+t701-t745+t9.*(t30-t150).*1.2516e-2+t271.*(t30-t150)).*(-1.0./2.0);
t2073 = t1996.*1.225946;
t2074 = t1995.*3.587895;
t2075 = t1996.*3.587895;
t2088 = t284+t589+t792+t919+t951+t1016;
t2092 = t177.*(t566+t678+t701-t745+t9.*(t30-t150).*1.2516e-2+t271.*(t30-t150)).*(-1.0./2.0);
t2095 = t2017.*1.666555;
t2096 = t2017.*1.225946;
t2097 = t2018.*1.225946;
t2099 = (t1640.*t1657)./2.0;
t2102 = t1995.*3.746479959e-1;
t2103 = t1996.*1.9076837715e-1;
t2120 = -t2117;
t2126 = (t1663.*t1671)./2.0;
t2133 = t290+t803+t810+t949+t961+t970;
t2137 = -t2136;
t2173 = t401+t785+t936+t955+t994+t1037;
t2175 = (t1680.*t1721)./2.0;
t2188 = t2018.*(-5.034347249e-2);
t2191 = t9.*t2087.*3.07985e-2;
t2193 = t2017.*(-1.4653732538e-2);
t2255 = (t1709.*t1802)./2.0;
t2273 = -t2267;
t2286 = (t1184.*t2087)./2.0;
t2302 = -t2301;
t2329 = -t7.*(-t98+t1575+t1995);
t2330 = -t15.*(-t98+t1575+t1995);
t2334 = t7.*(-t98+t1575+t1995);
t2335 = t15.*(-t98+t1575+t1995);
t2338 = -t2337;
t2339 = t91+t118+t1562+t1996;
t2354 = t1536+t1661+t1673;
t2359 = t374+t608+t802+t808+t1002+t1013+t1102+t1126;
t2364 = (t1483.*t2182)./2.0;
t2394 = (t1513.*t2182)./2.0;
t2418 = t13.*t2353.*1.24749e-1;
t2448 = t118+t156+t353+t531+t1562+t1996;
t2449 = t121+t138+t349+t487+t1575+t1995;
t2460 = (t1091.*t2353)./2.0;
t2536 = (t1897.*t2182)./2.0;
t2556 = (t221.*t2499)./2.0;
t2560 = (t582.*t2499)./2.0;
t2614 = (t1185.*t2499)./2.0;
t2781 = t979+t999+t1042+t1058+t1182+t1190+t1319+t1323+t1334+t1352+t1362;
t3081 = t1152+t1156+t1176+t1274+t1278+t1442+t1494+t1598+t1605+t1776+t1780+t1805+t1866;
t220 = t202.*(1.1e+1./1.25e+2);
t270 = -t227;
t313 = t9.*t238;
t317 = t17.*t238;
t648 = t152+t200;
t660 = t161+t202;
t819 = t202.*4.815e-3;
t821 = t202.*4.354e-3;
t826 = t202.*6.0149e-2;
t829 = t200.*1.0517e-2;
t830 = t202.*1.196e-3;
t831 = t202.*1.0517e-2;
t834 = t200.*1.158e-3;
t841 = t200.*1.964e-3;
t844 = t202.*4.252e-3;
t845 = t200.*1.4117e-2;
t850 = t202.*3.41e-4;
t854 = t202.*7.41e-4;
t857 = t202.*1.09e-4;
t864 = t200.*1.09e-4;
t878 = t234.*7.35522e-1;
t881 = t235.*7.35522e-1;
t883 = t227.*7.35522e-1;
t888 = t238.*1.666555;
t891 = t227.*1.666555;
t948 = t287.*7.35522e-1;
t953 = t293.*7.35522e-1;
t1048 = -t1043;
t1050 = -t1044;
t1139 = t8.*t1083;
t1141 = t16.*t1083;
t1163 = -t1151;
t1220 = t200.*2.3526756935e-2;
t1221 = t200.*1.7527158935e-2;
t1223 = t202.*1.7527158935e-2;
t1224 = t202.*3.127439544e-3;
t1225 = t202.*7.735484874e-3;
t1228 = t202.*1.00241616695e-1;
t1231 = -t1213;
t1232 = -t1214;
t1279 = t238.*2.3526756935e-2;
t1280 = t235.*3.127439544e-3;
t1282 = t234.*7.735484874e-3;
t1290 = t227.*1.00241616695e-1;
t1327 = t293.*3.127439544e-3;
t1328 = t287.*7.735484874e-3;
t1378 = -t1373;
t1380 = -t1374;
t1391 = t1088.*7.35522e-1;
t1392 = t1090.*7.35522e-1;
t1460 = -t1446;
t1468 = t200.*1.037589172186849e-4;
t1484 = t202.*9.3569097314605e-5;
t1488 = -t8.*(t116+t186+t776+t7.*(t131+t14.*t91));
t1489 = -t16.*(t116+t186+t776+t7.*(t131+t14.*t91));
t1500 = t9.*t1467;
t1501 = t17.*t1467;
t1503 = t1071.*(t149-t202).*(-1.0./2.0);
t1504 = t202.*4.909651967360946e-3;
t1509 = t1069.*(t149-t202).*(-1.0./2.0);
t1510 = (t1071.*(t149-t202))./2.0;
t1512 = (t1069.*(t149-t202))./2.0;
t1583 = t1444.*3.228604;
t1584 = t1446.*3.228604;
t1586 = t1446.*3.587895;
t1590 = -t1582;
t1594 = -t1587;
t1610 = t16.*(t116+t186+t776+t7.*(t131+t14.*t91)).*(-7.35522e-1);
t1611 = t8.*(t116+t186+t776+t7.*(t131+t14.*t91)).*(-1.666555);
t1612 = t16.*(t116+t186+t776+t7.*(t131+t14.*t91)).*(-1.666555);
t1618 = t238+t439+t508+t572;
t1637 = t1432.*(t149-t202).*(-1.0./2.0);
t1641 = (t1432.*(t149-t202))./2.0;
t1645 = t1441.*(t149-t202).*(-1.0./2.0);
t1650 = (t1441.*(t149-t202))./2.0;
t1715 = t8.*(t116+t186+t776+t7.*(t131+t14.*t91)).*(-2.3526756935e-2);
t1716 = t16.*(t116+t186+t776+t7.*(t131+t14.*t91)).*(-1.00241616695e-1);
t1717 = t8.*(t116+t186+t776+t7.*(t131+t14.*t91)).*2.3526756935e-2;
t1718 = t893.*t1467;
t1719 = t895.*t1467;
t1799 = t81+t132+t134+t506+t538+t720+t762;
t1838 = (t721.*t1682)./2.0;
t1841 = t1444+t1452;
t1845 = t15.*t1840;
t1847 = t7.*t1840;
t1848 = t14.*t1843;
t1849 = -t15.*(t1446+t5.*(t798-t806));
t1850 = t6.*t1843;
t1851 = -t7.*(t1446+t5.*(t798-t806));
t1855 = t7.*(t1446+t5.*(t798-t806));
t1862 = t1738.*(t149-t202).*(-1.0./2.0);
t1865 = (t1738.*(t149-t202))./2.0;
t1867 = -t1863;
t1870 = t1751.*(t149-t202).*(-1.0./2.0);
t1871 = t7.*t1711.*2.11820788799e-1;
t1875 = -t1869;
t1876 = (t1751.*(t149-t202))./2.0;
t1885 = t260+t467+t594+t625+t672+t768;
t1890 = -t1889;
t1893 = t460+t486+t577+t586+t736+t770;
t1896 = (t7.*(t260+t467-t585+t594-t667+t768))./2.0;
t1901 = (t8.*t1887)./2.0;
t1902 = (t14.*t15.*(t260+t467-t585+t594-t667+t768))./2.0;
t1903 = t334+t471+t595+t628+t771+t786;
t1907 = (t15.*t16.*t1887)./2.0;
t1908 = -t1904;
t1914 = -t1912;
t1915 = -t1913;
t1917 = (t8.*t1900)./2.0;
t1921 = (t16.*t1898)./2.0;
t1929 = (t6.*(t334+t471-t592+t595-t755+t786))./2.0;
t1933 = (t15.*t16.*t1900)./2.0;
t1935 = (t8.*t15.*t1898)./2.0;
t1940 = t15.*(t1446+t5.*(t798-t806)).*(-1.225946);
t1943 = (t13.*t14.*(t334+t471-t592+t595-t755+t786))./2.0;
t1951 = (t141.*(t260+t467-t585+t594-t667+t768))./2.0;
t1952 = t195+t211+t373+t503+t653+t715+t731;
t1959 = t106.*(t334+t471-t592+t595-t755+t786);
t1961 = -t1954;
t1964 = t193+t216+t421+t537+t647+t713+t729;
t1966 = (t108.*t1898)./2.0;
t1970 = (t142.*t1900)./2.0;
t1973 = (t176.*t1887)./2.0;
t1974 = -(t37-t163).*(t260+t467-t585+t594-t667+t768);
t1978 = (t37-t163).*(t260+t467-t585+t594-t667+t768);
t1982 = t1579+t1599;
t1984 = t1576+t1600;
t1986 = t1580+t1606;
t1992 = t875.*t1840;
t1997 = t880.*t1840;
t1999 = t15.*(t1446+t5.*(t798-t806)).*(-5.034347249e-2);
t2003 = t13.*t1840.*4.02765120396e-1;
t2008 = t5.*t1843.*4.02765120396e-1;
t2009 = t13.*(t1446+t5.*(t798-t806)).*(-4.02765120396e-1);
t2013 = t1887.*(t149-t202).*(-1.0./2.0);
t2016 = (t1887.*(t149-t202))./2.0;
t2024 = t615+t702+t726+t745+t814+t828;
t2028 = t1900.*(t149-t202).*(-1.0./2.0);
t2033 = t601+t711+t758+t767+t838+t846;
t2038 = (t8.*t2029)./2.0;
t2042 = (t15.*t16.*t2029)./2.0;
t2052 = (t1568.*t1678)./2.0;
t2053 = -t2049;
t2055 = (t1524.*t1723)./2.0;
t2068 = (t142.*t2029)./2.0;
t2078 = -t2073;
t2100 = -t2096;
t2101 = -t2097;
t2105 = -t2102;
t2107 = t7.*(t186-t373-t503+t646+t686+t776+t7.*(t131+t14.*t91)).*(-2.11820788799e-1);
t2127 = (t1663.*t1678)./2.0;
t2131 = t343+t809+t811+t916+t917+t956;
t2153 = (t1483.*t1840)./2.0;
t2154 = t2029.*(t149-t202).*(-1.0./2.0);
t2162 = t1483.*(t1446+t5.*(t798-t806)).*(-1.0./2.0);
t2170 = (t1662.*t1723)./2.0;
t2177 = (t1682.*t1721)./2.0;
t2178 = -t2175;
t2179 = (t1513.*t1840)./2.0;
t2185 = t1513.*(t1446+t5.*(t798-t806)).*(-1.0./2.0);
t2192 = t17.*t2088.*3.07985e-2;
t2195 = -t2191;
t2197 = (t1533.*t1840)./2.0;
t2201 = t1533.*(t1446+t5.*(t798-t806)).*(-1.0./2.0);
t2203 = (t1533.*(t1446+t5.*(t798-t806)))./2.0;
t2204 = (t1536.*t1843)./2.0;
t2220 = (t1524.*t1879)./2.0;
t2234 = t15.*t2133.*1.727815e-1;
t2252 = (t1711.*t1796)./2.0;
t2259 = t305+t476+t488+t984+t1024+t1117+t1157;
t2283 = (t1186.*t2088)./2.0;
t2297 = (t1662.*t1879)./2.0;
t2314 = (t1056.*t2173)./2.0;
t2321 = (t1189.*t2173)./2.0;
t2326 = t98+t1563+t2000;
t2332 = (t1383.*t2133)./2.0;
t2343 = t8.*t2339;
t2344 = t16.*t2339;
t2352 = t801+t836+t908+t982+t1039+t1104+t1155;
t2355 = t800+t852+t925+t1021+t1023+t1101+t1154;
t2360 = t2335.*(-1.666555);
t2361 = t2334.*(-1.225946);
t2362 = t2335.*(-1.225946);
t2363 = t2335.*1.225946;
t2368 = -t2364;
t2374 = t1796.*(t186-t373-t503+t646+t686+t776+t7.*(t131+t14.*t91)).*(-1.0./2.0);
t2390 = (t1840.*t1897)./2.0;
t2400 = -t2394;
t2403 = t1897.*(t1446+t5.*(t798-t806)).*(-1.0./2.0);
t2410 = (t1897.*(t1446+t5.*(t798-t806)))./2.0;
t2419 = t7.*(t796-t908-t982+t1018+t1086-t1155+t7.*(t131+t14.*t91).*1.225946).*(-1.727815e-1);
t2420 = -t2418;
t2425 = t2334.*(-5.034347249e-2);
t2427 = t2335.*(-1.4653732538e-2);
t2429 = t2335.*1.4653732538e-2;
t2434 = t890.*t2339;
t2435 = t899.*t2339;
t2468 = (t1056.*t2359)./2.0;
t2472 = (t1189.*t2359)./2.0;
t2478 = t1379.*(t796-t908-t982+t1018+t1086-t1155+t7.*(t131+t14.*t91).*1.225946).*(-1.0./2.0);
t2511 = t6.*t2449.*4.9251034665e-2;
t2512 = t14.*t2448.*4.9251034665e-2;
t2516 = (t1879.*t2173)./2.0;
t2558 = -t2556;
t2561 = -t2560;
t2562 = t81+t132+t506+t538+t720+t762+t1574+t2001;
t2589 = t1711.*(t796-t908-t982+t1018+t1086-t1155+t7.*(t131+t14.*t91).*1.225946).*(-1.0./2.0);
t2593 = (t1711.*(t796-t908-t982+t1018+t1086-t1155+t7.*(t131+t14.*t91).*1.225946))./2.0;
t2608 = (t1723.*t2359)./2.0;
t2623 = (t1840.*t2353)./2.0;
t2626 = t2353.*(t1446+t5.*(t798-t806)).*(-1.0./2.0);
t2628 = (t2353.*(t1446+t5.*(t798-t806)))./2.0;
t2629 = t1843.*(-t872+t1017+t1573.*3.228604+t1654).*(-1.0./2.0);
t2630 = t650+t656+t903+t973+t1676+t2074;
t2631 = t634+t658+t904+t993+t1668+t2075;
t2641 = (t1727.*t2448)./2.0;
t2642 = (t1728.*t2449)./2.0;
t2684 = (t1906.*t2449)./2.0;
t2687 = (t1911.*t2448)./2.0;
t2708 = t119+t773+t2017+t2330;
t2709 = t116+t776+t2018+t2334;
t2710 = -t9.*(t97+t729+t2022+t2335);
t2711 = -t17.*(t97+t729+t2022+t2335);
t2714 = t17.*(t97+t729+t2022+t2335);
t2719 = (t1840.*t2499)./2.0;
t2721 = t2499.*(t1446+t5.*(t798-t806)).*(-1.0./2.0);
t2723 = (t2499.*(t1446+t5.*(t798-t806)))./2.0;
t2735 = t9.*(t97+t729+t2022+t2335).*(-7.35522e-1);
t2751 = t9.*(t97+t729+t2022+t2335).*(-7.735484874e-3);
t2754 = t893.*(t97+t729+t2022+t2335);
t2755 = t895.*(t97+t729+t2022+t2335);
t2815 = t373+t503+t653+t715+t731+t2023+t2329;
t2816 = t421+t537+t647+t713+t729+t2022+t2335;
t2922 = t7.*(-t908-t982+t1018+t1086-t1155+t2097+t2334.*1.225946).*(-1.727815e-1);
t2938 = t1379.*(-t908-t982+t1018+t1086-t1155+t2097+t2334.*1.225946).*(-1.0./2.0);
t2963 = t1711.*(-t908-t982+t1018+t1086-t1155+t2097+t2334.*1.225946).*(-1.0./2.0);
t2964 = (t1711.*(-t908-t982+t1018+t1086-t1155+t2097+t2334.*1.225946))./2.0;
t2984 = ((t186-t373-t503+t646+t686+t776+t7.*(t131+t14.*t91)).*(-t908-t982+t1018+t1086-t1155+t2097+t2334.*1.225946))./2.0;
t437 = -t313;
t665 = t9.*t648;
t666 = t17.*t648;
t799 = t175+t220;
t815 = -t9.*(t172-t220);
t816 = -t17.*(t172-t220);
t823 = t9.*(t172-t220);
t825 = -t819;
t835 = -t821;
t843 = -t826;
t848 = -t830;
t849 = -t831;
t866 = -t857;
t907 = -t883;
t915 = -t891;
t928 = t313.*7.35522e-1;
t931 = t317.*7.35522e-1;
t1133 = t322.*t648;
t1136 = t271.*t648;
t1210 = t17.*(t172-t220).*(-7.35522e-1);
t1237 = -t1223;
t1238 = -t1225;
t1240 = -t1228;
t1297 = -t1280;
t1301 = -t1282;
t1309 = -t1290;
t1314 = t313.*3.127439544e-3;
t1321 = t317.*7.735484874e-3;
t1412 = t1141.*7.35522e-1;
t1414 = t1139.*1.666555;
t1416 = t1141.*1.666555;
t1449 = t323+t1139;
t1471 = -t9.*(t239-t1139);
t1473 = -t17.*(t239-t1139);
t1478 = -t1468;
t1480 = t17.*(t172-t220).*(-3.127439544e-3);
t1490 = t17.*(t239-t1139);
t1493 = -t1484;
t1499 = (t648.*t1076)./2.0;
t1556 = t1141.*1.00241616695e-1;
t1557 = t1139.*2.3526756935e-2;
t1591 = -t1584;
t1593 = -t1586;
t1603 = t9.*(t239-t1139).*(-7.35522e-1);
t1614 = t1500.*7.35522e-1;
t1615 = t1501.*7.35522e-1;
t1617 = t270+t366+t454+t561;
t1638 = t570+t1488;
t1639 = (t648.*t1440)./2.0;
t1703 = t9.*(t239-t1139).*(-3.127439544e-3);
t1807 = t8.*t1618.*8.7635794675e-3;
t1823 = t79+t270+t550+t573+t689+t727;
t1842 = t1450+t1460;
t1844 = t14.*t1841;
t1846 = t6.*t1841;
t1852 = -t1847;
t1873 = (t648.*t1757)./2.0;
t1877 = -t1871;
t1899 = -t1896;
t1905 = -t1902;
t1909 = (t15.*t1893)./2.0;
t1910 = t205+t234+t317+t445+t482+t618+t682;
t1916 = (t7.*t14.*t1893)./2.0;
t1922 = t1847.*1.666555;
t1923 = t1847.*1.225946;
t1925 = t1845.*1.225946;
t1928 = -t1917;
t1930 = -t1921;
t1934 = t1850.*3.587895;
t1936 = t1848.*3.587895;
t1937 = t1855.*(-1.666555);
t1938 = t1855.*(-1.225946);
t1939 = t1848.*1.225946;
t1941 = -t1933;
t1942 = t888+t941+t980+t1001;
t1946 = t1855.*1.666555;
t1947 = t1855.*1.225946;
t1948 = -t1943;
t1953 = (t107.*t1893)./2.0;
t1963 = t1850.*3.746479959e-1;
t1965 = t1848.*1.9076837715e-1;
t1969 = -t1966;
t1971 = -t1970;
t1972 = t237+t357+t541+t583+t724+t1141;
t1975 = -t1973;
t1976 = t187.*t1893;
t1983 = t1583+t1588;
t2002 = t5.*t1841.*4.02765120396e-1;
t2004 = t1855.*(-1.4653732538e-2);
t2011 = -t2008;
t2025 = (t648.*t1898)./2.0;
t2030 = t480+t708+t751+t760+t834+t850;
t2040 = -t2038;
t2044 = -t2042;
t2046 = (t9.*t2033)./2.0;
t2051 = (t16.*t17.*t2033)./2.0;
t2057 = -t2052;
t2070 = -t2068;
t2072 = (t109.*t2033)./2.0;
t2079 = (t221.*t1984)./2.0;
t2082 = t221.*(t1586+t5.*(t798-t806).*3.587895).*(-1.0./2.0);
t2086 = t13.*t1982.*1.24749e-1;
t2089 = t5.*t1986.*1.24749e-1;
t2091 = t13.*(t1584+t5.*(t798-t806).*3.228604).*(-1.24749e-1);
t2106 = (t582.*t1984)./2.0;
t2109 = t582.*(t1586+t5.*(t798-t806).*3.587895).*(-1.0./2.0);
t2116 = t2033.*(t41-t154).*(-1.0./2.0);
t2119 = t15.*t1964.*2.11820788799e-1;
t2129 = -t2127;
t2146 = (t1535.*t1799)./2.0;
t2147 = t1461+t1848;
t2156 = t1477+t1850;
t2160 = t65+t128+t237+t741+t750+t832+t856+t1141;
t2167 = t540+t638+t703+t717+t829+t1489;
t2180 = (t1618.*t1784)./2.0;
t2181 = -t2177;
t2198 = -t2197;
t2199 = (t1536.*t1841)./2.0;
t2205 = (t1091.*t1982)./2.0;
t2208 = t1091.*(t1584+t5.*(t798-t806).*3.228604).*(-1.0./2.0);
t2209 = (t1107.*t1986)./2.0;
t2210 = (t1091.*(t1584+t5.*(t798-t806).*3.228604))./2.0;
t2213 = (t1636.*t1799)./2.0;
t2214 = (t1185.*t1984)./2.0;
t2218 = t1185.*(t1586+t5.*(t798-t806).*3.587895).*(-1.0./2.0);
t2221 = (t1185.*(t1586+t5.*(t798-t806).*3.587895))./2.0;
t2222 = -t2220;
t2231 = t7.*t2131.*1.727815e-1;
t2237 = -t2234;
t2254 = -t2252;
t2300 = -t2297;
t2306 = t8.*(-t551-t570+t723+t742+t831+t8.*(t116+t186+t776+t7.*(t131+t14.*t91))).*(-8.7635794675e-3);
t2327 = (t1379.*t2131)./2.0;
t2345 = -t2343;
t2346 = -t2344;
t2347 = (t1524.*(t676+t692-t826+t845-t1467))./2.0;
t2365 = (t1109.*t2259)./2.0;
t2366 = (t1119.*t2259)./2.0;
t2396 = -t2390;
t2398 = t2343.*7.35522e-1;
t2399 = t2343.*1.666555;
t2401 = t2344.*1.666555;
t2402 = (t1802.*t1964)./2.0;
t2417 = (t1662.*(t676+t692-t826+t845-t1467))./2.0;
t2422 = t15.*t2355.*1.727815e-1;
t2436 = t2344.*(-2.3526756935e-2);
t2437 = t2343.*(-1.00241616695e-1);
t2442 = t1035+t1050+t1093+t1137+t1221+t1612;
t2469 = -t2468;
t2473 = -t2472;
t2474 = t8.*(-t996-t1045+t1127+t1148+t1223+t8.*(t116+t186+t776+t7.*(t131+t14.*t91)).*1.666555).*(-5.2585e-3);
t2476 = t1784.*(-t551-t570+t723+t742+t831+t8.*(t116+t186+t776+t7.*(t131+t14.*t91))).*(-1.0./2.0);
t2479 = (t1383.*t2355)./2.0;
t2494 = (t1725.*t2259)./2.0;
t2495 = (t1799.*t2211)./2.0;
t2518 = -t2516;
t2531 = t2131.*(t186-t373-t503+t646+t686+t776+t7.*(t131+t14.*t91)).*(-1.0./2.0);
t2533 = (t2131.*(t186-t373-t503+t646+t686+t776+t7.*(t131+t14.*t91)))./2.0;
t2541 = (t1964.*t2133)./2.0;
t2551 = t1265.*(-t996-t1045+t1127+t1148+t1223+t8.*(t116+t186+t776+t7.*(t131+t14.*t91)).*1.666555).*(-1.0./2.0);
t2565 = (t1982.*t2149)./2.0;
t2568 = t2149.*(t1584+t5.*(t798-t806).*3.228604).*(-1.0./2.0);
t2570 = (t2149.*(t1584+t5.*(t798-t806).*3.228604))./2.0;
t2578 = t1986.*(-t1107+t1550+t1573).*(-1.0./2.0);
t2595 = (t1709.*t2355)./2.0;
t2596 = (t1984.*t2182)./2.0;
t2601 = t2182.*(t1586+t5.*(t798-t806).*3.587895).*(-1.0./2.0);
t2604 = (t2182.*(t1586+t5.*(t798-t806).*3.587895))./2.0;
t2612 = -t2608;
t2615 = t1618.*(-t996-t1045+t1127+t1148+t1223+t8.*(t116+t186+t776+t7.*(t131+t14.*t91)).*1.666555).*(-1.0./2.0);
t2618 = (t1618.*(-t996-t1045+t1127+t1148+t1223+t8.*(t116+t186+t776+t7.*(t131+t14.*t91)).*1.666555))./2.0;
t2622 = (t2173.*(t676+t692-t826+t845-t1467))./2.0;
t2625 = -t2623;
t2627 = t1841.*(-t872+t1017+t1573.*3.228604+t1654).*(-1.0./2.0);
t2648 = t6.*t2630.*1.3727e-2;
t2649 = t14.*t2631.*1.3727e-2;
t2673 = (t1535.*t2562)./2.0;
t2676 = (t1064.*t2630)./2.0;
t2677 = (t1063.*t2631)./2.0;
t2685 = (t1636.*t2562)./2.0;
t2696 = (t2359.*(t676+t692-t826+t845-t1467))./2.0;
t2712 = t8.*t2709;
t2713 = t16.*t2709;
t2720 = -t2719;
t2727 = (t1454.*t2630)./2.0;
t2731 = (t1465.*t2631)./2.0;
t2736 = t2714.*(-7.35522e-1);
t2740 = t2714.*7.35522e-1;
t2744 = t305+t488+t984+t1024+t1117+t1157+t1677+t2078;
t2750 = t2714.*(-3.127439544e-3);
t2841 = (t2211.*t2562)./2.0;
t2843 = t7.*t2815.*2.11820788799e-1;
t2844 = t15.*t2816.*2.11820788799e-1;
t2851 = (t2259.*t2562)./2.0;
t2914 = t908+t982+t1039+t1104+t1155+t2101+t2361;
t2915 = t925+t1021+t1023+t1101+t1154+t2100+t2363;
t2917 = (t1796.*t2815)./2.0;
t2919 = (t1802.*t2816)./2.0;
t2951 = (t2131.*t2815)./2.0;
t2953 = (t2133.*t2816)./2.0;
t2983 = t2815.*(t796-t908-t982+t1018+t1086-t1155+t7.*(t131+t14.*t91).*1.225946).*(-1.0./2.0);
t2985 = (t2355.*t2816)./2.0;
t3195 = t963+t989+t1040+t1047+t1168+t1234+t1235+t1289+t1315+t1330+t1747+t1765+t1829+t1833+t2138+t2192+t2195+t2342;
t3213 = t1166+t1170+t1178+t1260+t1293+t1487+t1498+t1505+t1516+t1530+t1631+t1634+t1754+t1763+t1777+t1812+t1864+t1868+t1874+t2064+t2098+t2099+t2283+t2286+t2341;
t679 = -t666;
t969 = -t928;
t1078 = t210+t665;
t1085 = t665.*1.2516e-2;
t1123 = t665.*6.1597e-2;
t1125 = t666.*6.1597e-2;
t1130 = t665.*4.252e-3;
t1135 = t665.*1.196e-3;
t1140 = t666.*1.0517e-2;
t1145 = t666.*1.0027e-2;
t1159 = t666.*7.41e-4;
t1209 = t823.*(-7.35522e-1);
t1227 = t823.*7.35522e-1;
t1337 = -t1321;
t1389 = t665.*4.5305948634e-2;
t1390 = t666.*4.5305948634e-2;
t1401 = t665.*3.127439544e-3;
t1402 = t666.*7.735484874e-3;
t1481 = t823.*(-7.735484874e-3);
t1543 = t665.*1.672482661783778e-3;
t1546 = t666.*5.48359106408232e-4;
t1559 = -t1556;
t1604 = t1490.*(-7.35522e-1);
t1608 = t1490.*7.35522e-1;
t1623 = ((t666+t9.*(t37-t163)).*(t271-t298))./2.0;
t1642 = -t1639;
t1646 = t9.*t1638;
t1647 = t17.*t1638;
t1704 = t1490.*(-7.735484874e-3);
t1710 = t1490.*7.735484874e-3;
t1740 = t1439.*(t666+t9.*(t37-t163)).*(-1.0./2.0);
t1741 = (t1439.*(t666+t9.*(t37-t163)))./2.0;
t1806 = t16.*t1617.*8.7635794675e-3;
t1809 = -t1807;
t1918 = t1846.*3.587895;
t1919 = t1844.*3.587895;
t1924 = t1844.*1.225946;
t1926 = t206+t235+t426+t437+t526+t607+t683;
t1927 = -t1916;
t1931 = -t1922;
t1932 = -t1923;
t1945 = t915+t939+t958+t995;
t1956 = -t1953;
t1957 = t1846.*3.746479959e-1;
t1960 = t1844.*1.9076837715e-1;
t1967 = t1743.*(t666+t9.*(t37-t163)).*(-1.0./2.0);
t1968 = -t1965;
t1977 = t502+t552+t571+t704+t1449;
t1979 = -t1976;
t1985 = t1585+t1591;
t1988 = t1581+t1593;
t2005 = -t2002;
t2019 = t8.*t1942.*5.2585e-3;
t2027 = -t2025;
t2035 = t518+t687+t743+t778+t841+t866;
t2036 = t641+t680+t746+t769+t835+t864;
t2039 = (t7.*t2030)./2.0;
t2043 = (t14.*t15.*t2030)./2.0;
t2050 = -t2046;
t2069 = t17.*t1910.*2.2652974317e-2;
t2071 = (t141.*t2030)./2.0;
t2077 = -t2072;
t2085 = t5.*t1983.*1.24749e-1;
t2093 = -t2089;
t2094 = t119+t185+t212+t676+t692+t773+t843+t845;
t2104 = -t2030.*(t37-t163);
t2108 = t2030.*(t37-t163);
t2112 = t1894.*(t666+t9.*(t37-t163)).*(-1.0./2.0);
t2115 = (t1894.*(t666+t9.*(t37-t163)))./2.0;
t2121 = -t2119;
t2124 = t16.*t1972.*8.7635794675e-3;
t2135 = t1448+t1846;
t2139 = t1462+t1844;
t2150 = -t8.*(t1447-t1844);
t2152 = -t16.*(t1447-t1844);
t2159 = t8.*t2147;
t2161 = t16.*t2147;
t2166 = t7.*t2156;
t2168 = t15.*t2156;
t2172 = t551+t698+t764+t849+t1638;
t2176 = (t1537.*t1823)./2.0;
t2183 = -t2180;
t2184 = (t1617.*t1789)./2.0;
t2189 = (t1265.*t1942)./2.0;
t2206 = (t1107.*t1983)./2.0;
t2207 = -t2205;
t2216 = -t2213;
t2217 = -t2214;
t2228 = t8.*(t1447-t1844).*(-7.35522e-1);
t2229 = t8.*(t1447-t1844).*(-1.666555);
t2230 = t16.*(t1447-t1844).*(-1.666555);
t2232 = -t2231;
t2242 = (t1649.*t1823)./2.0;
t2244 = t2033.*(t666+t9.*(t37-t163)).*(-1.0./2.0);
t2245 = (t2033.*(t666+t9.*(t37-t163)))./2.0;
t2248 = t394+t907+t1006+t1009+t1115+t1120;
t2271 = t1595+t1939;
t2272 = t1601+t1936;
t2277 = t1607+t1934;
t2279 = t14.*(t1447-t1844).*(-4.9251034665e-2);
t2280 = t16.*(t1447-t1844).*(-2.3526756935e-2);
t2282 = t8.*(t1447-t1844).*(-1.00241616695e-1);
t2285 = t14.*(t1447-t1844).*4.9251034665e-2;
t2287 = t14.*t2147.*4.9251034665e-2;
t2288 = t890.*t2147;
t2289 = t899.*t2147;
t2294 = t6.*t2156.*4.9251034665e-2;
t2304 = t16.*t2167.*8.7635794675e-3;
t2307 = t293+t546+t690+t759+t840+t1090+t1471;
t2308 = t287+t571+t704+t733+t837+t1088+t1490;
t2311 = (t1657.*t1910)./2.0;
t2328 = -t2327;
t2331 = t886+t954+t1005+t1036+t1128+t1416;
t2333 = t910+t977+t997+t1000+t1094+t1414;
t2348 = t818+t878+t931+t944+t990+t1032+t1087;
t2369 = -t2366;
t2373 = t1535.*(t1447-t1844).*(-1.0./2.0);
t2375 = (t1789.*t1972)./2.0;
t2378 = (t1535.*t2147)./2.0;
t2405 = (t1537.*t2160)./2.0;
t2406 = -t2398;
t2407 = -t2399;
t2408 = -t2401;
t2424 = -t2422;
t2426 = t1636.*(t1447-t1844).*(-1.0./2.0);
t2428 = (t1636.*(t1447-t1844))./2.0;
t2430 = (t1636.*t2147)./2.0;
t2432 = (t1649.*t2160)./2.0;
t2443 = t996+t1045+t1111+t1160+t1237+t1611;
t2452 = t1727.*(t1447-t1844).*(-1.0./2.0);
t2453 = (t1727.*(t1447-t1844))./2.0;
t2454 = (t1727.*t2147)./2.0;
t2456 = (t1728.*t2156)./2.0;
t2471 = t563+t793+t833+t1100+t1113+t1163+t1220+t1240;
t2475 = (t1789.*t2167)./2.0;
t2477 = t16.*t2442.*5.2585e-3;
t2481 = t462+t627+t882+t1131+t1132+t1226+t1236+t1412;
t2493 = (t1910.*t2088)./2.0;
t2513 = (t1823.*t2219)./2.0;
t2522 = t1911.*(t1447-t1844).*(-1.0./2.0);
t2523 = (t1911.*(t1447-t1844))./2.0;
t2524 = (t1911.*t2147)./2.0;
t2525 = (t1906.*t2156)./2.0;
t2547 = t1942.*(-t551-t570+t723+t742+t831+t8.*(t116+t186+t776+t7.*(t131+t14.*t91))).*(-1.0./2.0);
t2549 = (t1942.*(-t551-t570+t723+t742+t831+t8.*(t116+t186+t776+t7.*(t131+t14.*t91))))./2.0;
t2550 = (t1263.*t2442)./2.0;
t2554 = t953+t1003+t1095+t1138+t1212+t1392+t1603;
t2567 = -t2565;
t2572 = t1983.*(-t1107+t1550+t1573).*(-1.0./2.0);
t2600 = -t2596;
t2617 = (t1617.*t2442)./2.0;
t2640 = t2211.*(t1447-t1844).*(-1.0./2.0);
t2643 = (t2147.*t2211)./2.0;
t2645 = (t2160.*t2219)./2.0;
t2658 = t2259.*(t1447-t1844).*(-1.0./2.0);
t2665 = (t2147.*t2259)./2.0;
t2686 = -t2685;
t2698 = (t1972.*t2442)./2.0;
t2699 = -t2696;
t2715 = -t2713;
t2737 = t2712.*1.666555;
t2738 = t2713.*1.666555;
t2739 = t2713.*7.35522e-1;
t2752 = t2713.*1.00241616695e-1;
t2753 = t2712.*2.3526756935e-2;
t2789 = (t1109.*t2744)./2.0;
t2792 = (t1119.*t2744)./2.0;
t2842 = t676+t692+t843+t845+t2708;
t2845 = -t2844;
t2853 = (t1725.*t2744)./2.0;
t2874 = t2631.*(t1447-t1844).*(-1.0./2.0);
t2876 = (t2631.*(t1447-t1844))./2.0;
t2878 = (t2147.*t2631)./2.0;
t2882 = (t2156.*t2630)./2.0;
t2887 = (t1799.*t2744)./2.0;
t2923 = t15.*t2915.*1.727815e-1;
t2927 = t2744.*(t1447-t1844).*(-1.0./2.0);
t2929 = (t2147.*t2744)./2.0;
t2937 = t563+t1100+t1113+t1163+t1220+t1240+t2095+t2360;
t2939 = (t1383.*t2915)./2.0;
t2941 = t2346+t2712;
t2943 = -t9.*(t2344-t2712);
t2944 = -t17.*(t2344-t2712);
t2949 = t9.*(t2344-t2712).*(-7.35522e-1);
t2950 = t17.*(t2344-t2712).*(-7.35522e-1);
t2952 = -t2951;
t2959 = t9.*(t2344-t2712).*(-3.127439544e-3);
t2960 = t17.*(t2344-t2712).*(-7.735484874e-3);
t2961 = t17.*(t2344-t2712).*7.735484874e-3;
t2965 = (t1709.*t2915)./2.0;
t2986 = (t1964.*t2915)./2.0;
t1097 = t209+t679;
t1143 = -t1123;
t1146 = -t1125;
t1153 = -t1140;
t1165 = -t1159;
t1397 = -t1389;
t1398 = -t1390;
t1409 = -t1402;
t1547 = -t1543;
t1609 = (t1052.*t1078)./2.0;
t1651 = -t1646;
t1726 = (t1078.*t1418)./2.0;
t1736 = t1646.*7.35522e-1;
t1737 = t1647.*7.35522e-1;
t1831 = t1646.*3.127439544e-3;
t1832 = t1647.*7.735484874e-3;
t1949 = (t1078.*t1729)./2.0;
t1962 = -t1960;
t2020 = t16.*t1945.*5.2585e-3;
t2021 = -t2019;
t2041 = -t2039;
t2045 = -t2043;
t2047 = (t8.*t2036)./2.0;
t2048 = (t16.*t2035)./2.0;
t2054 = (t15.*t16.*t2036)./2.0;
t2056 = (t8.*t15.*t2035)./2.0;
t2076 = (t108.*t2035)./2.0;
t2080 = t9.*t1926.*2.2652974317e-2;
t2081 = (t1078.*t1883)./2.0;
t2083 = (t142.*t2036)./2.0;
t2090 = -t2085;
t2111 = (t176.*t2036)./2.0;
t2118 = t2035.*(t30-t150).*(-1.0./2.0);
t2125 = -t2124;
t2130 = t8.*t1977.*8.7635794675e-3;
t2142 = t7.*t2135;
t2144 = t15.*t2135;
t2155 = t648.*t2035;
t2163 = -t2036.*(t149-t202);
t2169 = t2036.*(t149-t202);
t2190 = (t1263.*t1945)./2.0;
t2194 = -t2189;
t2226 = t1078.*(t566+t678+t701-t745+t9.*(t30-t150).*1.2516e-2+t271.*(t30-t150)).*(-1.0./2.0);
t2227 = t695+t820+t848+t869+t1085+t1136;
t2233 = t2159.*7.35522e-1;
t2235 = t2159.*1.666555;
t2236 = t2161.*1.666555;
t2238 = t2168.*1.225946;
t2240 = t2168.*1.666555;
t2241 = t2166.*1.225946;
t2246 = t761+t854+t858+t867+t1133+t1145;
t2249 = t8.*(-t673+t819-t1135+t1159+t277.*(t37-t163)+t361.*(t37-t163)).*(-1.0./2.0);
t2250 = t15.*t16.*(-t673+t819-t1135+t1159+t277.*(t37-t163)+t361.*(t37-t163)).*(-1.0./2.0);
t2258 = t142.*(-t673+t819-t1135+t1159+t277.*(t37-t163)+t361.*(t37-t163)).*(-1.0./2.0);
t2262 = t1589+t1918;
t2264 = t1590+t1924;
t2265 = t1594+t1919;
t2268 = t176.*(-t673+t819-t1135+t1159+t277.*(t37-t163)+t361.*(t37-t163)).*(-1.0./2.0);
t2270 = t6.*t2135.*4.9251034665e-2;
t2274 = (t176.*(-t673+t819-t1135+t1159+t277.*(t37-t163)+t361.*(t37-t163)))./2.0;
t2291 = -t2287;
t2292 = t2166.*5.034347249e-2;
t2293 = t2168.*1.4653732538e-2;
t2299 = -t2294;
t2310 = (t149-t202).*(-t673+t819-t1135+t1159+t277.*(t37-t163)+t361.*(t37-t163));
t2315 = (t1658.*t1926)./2.0;
t2319 = t14.*(t1587-t1919).*(-1.3727e-2);
t2320 = t14.*(t1587-t1919).*1.3727e-2;
t2322 = t14.*t2272.*1.3727e-2;
t2323 = t6.*t2277.*1.3727e-2;
t2349 = t813+t881+t938+t969+t1019+t1030+t1089;
t2356 = t2248.*(t385-t428).*(-1.0./2.0);
t2357 = (t1134.*t2248)./2.0;
t2370 = t1063.*(t1587-t1919).*(-1.0./2.0);
t2372 = (t1063.*(t1587-t1919))./2.0;
t2376 = (t1063.*t2272)./2.0;
t2377 = -t2375;
t2380 = t16.*t2331.*5.2585e-3;
t2381 = t8.*t2333.*5.2585e-3;
t2382 = t9.*t2307.*2.2652974317e-2;
t2384 = (t1784.*t1977)./2.0;
t2385 = (t1064.*t2277)./2.0;
t2386 = t17.*t2308.*2.2652974317e-2;
t2388 = t1109.*(t1582-t1924).*(-1.0./2.0);
t2391 = t1119.*(t1582-t1924).*(-1.0./2.0);
t2397 = (t1119.*(t1582-t1924))./2.0;
t2409 = (t1109.*t2271)./2.0;
t2411 = (t1119.*t2271)./2.0;
t2412 = -t2405;
t2414 = t17.*t2348.*3.07985e-2;
t2431 = -t2430;
t2433 = -t2432;
t2440 = t1465.*(t1587-t1919).*(-1.0./2.0);
t2441 = (t1465.*(t1587-t1919))./2.0;
t2444 = (t1454.*t2277)./2.0;
t2446 = (t1465.*t2272)./2.0;
t2450 = (t1728.*t2135)./2.0;
t2455 = -t2454;
t2457 = -t2456;
t2458 = (t1945.*t1972)./2.0;
t2461 = (t1942.*t1977)./2.0;
t2462 = (t1263.*t2331)./2.0;
t2463 = (t1265.*t2333)./2.0;
t2467 = (t1186.*t2348)./2.0;
t2480 = (t1722.*t2248)./2.0;
t2488 = t1845+t2166;
t2492 = t1852+t2168;
t2500 = (t1926.*t2087)./2.0;
t2502 = -t9.*(t1847-t2168);
t2503 = -t17.*(t1847-t2168);
t2504 = (t1658.*t2307)./2.0;
t2505 = t17.*(t1847-t2168);
t2507 = (t1657.*t2308)./2.0;
t2508 = t1725.*(t1582-t1924).*(-1.0./2.0);
t2510 = (t1725.*t2271)./2.0;
t2514 = (t1618.*t2333)./2.0;
t2515 = (t1617.*t2331)./2.0;
t2519 = (t1906.*t2135)./2.0;
t2521 = t1537.*(t111-t181+t560-t1130+t1140+t275.*(t37-t163)+t315.*(t37-t163)+t16.*(t116+t186+t776+t7.*(t131+t14.*t91))).*(-1.0./2.0);
t2526 = -t2524;
t2527 = -t2525;
t2543 = t9.*(t1847-t2168).*(-7.35522e-1);
t2545 = (t1945.*t2167)./2.0;
t2548 = t1799.*(t1582-t1924).*(-1.0./2.0);
t2552 = (t1640.*t2348)./2.0;
t2555 = t948+t1007+t1098+t1122+t1229+t1391+t1608;
t2557 = (t1799.*t2271)./2.0;
t2559 = (t1056.*t2471)./2.0;
t2563 = t1649.*(t111-t181+t560-t1130+t1140+t275.*(t37-t163)+t315.*(t37-t163)+t16.*(t116+t186+t776+t7.*(t131+t14.*t91))).*(-1.0./2.0);
t2571 = (t1189.*t2471)./2.0;
t2583 = t9.*(t688-t844+t1125-t1501+t1646+t9.*(t37-t163).*6.1597e-2+t17.*(t172-t220)).*(-2.2652974317e-2);
t2598 = t9.*(t1847-t2168).*(-7.735484874e-3);
t2599 = t15.*(t1847-t2168).*(-2.11820788799e-1);
t2602 = t893.*(t1847-t2168);
t2603 = t895.*(t1847-t2168);
t2605 = t2481.*(t385-t428).*(-1.0./2.0);
t2606 = t9.*t2554.*3.07985e-2;
t2609 = (t2481.*(t385-t428))./2.0;
t2611 = (t1134.*t2481)./2.0;
t2633 = (t1184.*t2554)./2.0;
t2638 = t1524.*(t1847-t2168).*(-1.0./2.0);
t2646 = -t2645;
t2650 = (t1723.*t2471)./2.0;
t2651 = (t2160.*t2248)./2.0;
t2657 = (t2087.*t2307)./2.0;
t2661 = (t2088.*t2308)./2.0;
t2666 = t1658.*(t688-t844+t1125-t1501+t1646+t9.*(t37-t163).*6.1597e-2+t17.*(t172-t220)).*(-1.0./2.0);
t2668 = (t1658.*(t688-t844+t1125-t1501+t1646+t9.*(t37-t163).*6.1597e-2+t17.*(t172-t220)))./2.0;
t2670 = t1662.*(t1847-t2168).*(-1.0./2.0);
t2671 = (t1722.*t2481)./2.0;
t2674 = ((t385-t428).*(t587-t756+t1043-t1401+t1402+t893.*(t37-t163)+t895.*(t37-t163)+t16.*(t116+t186+t776+t7.*(t131+t14.*t91)).*7.35522e-1))./2.0;
t2675 = t1134.*(t587-t756+t1043-t1401+t1402+t893.*(t37-t163)+t895.*(t37-t163)+t16.*(t116+t186+t776+t7.*(t131+t14.*t91)).*7.35522e-1).*(-1.0./2.0);
t2680 = (t1635.*t2554)./2.0;
t2692 = (t1823.*t2481)./2.0;
t2693 = t1802.*(t1847-t2168).*(-1.0./2.0);
t2695 = (t1802.*(t1847-t2168))./2.0;
t2697 = (t1879.*t2471)./2.0;
t2701 = -t2698;
t2702 = (t2167.*t2331)./2.0;
t2704 = t2333.*(-t551-t570+t723+t742+t831+t8.*(t116+t186+t776+t7.*(t131+t14.*t91))).*(-1.0./2.0);
t2705 = (t2333.*(-t551-t570+t723+t742+t831+t8.*(t116+t186+t776+t7.*(t131+t14.*t91))))./2.0;
t2706 = t1977.*(-t996-t1045+t1127+t1148+t1223+t8.*(t116+t186+t776+t7.*(t131+t14.*t91)).*1.666555).*(-1.0./2.0);
t2707 = (t1977.*(-t996-t1045+t1127+t1148+t1223+t8.*(t116+t186+t776+t7.*(t131+t14.*t91)).*1.666555))./2.0;
t2741 = -t2738;
t2742 = -t2739;
t2743 = t2219.*(t111-t181+t560-t1130+t1140+t275.*(t37-t163)+t315.*(t37-t163)+t16.*(t116+t186+t776+t7.*(t131+t14.*t91))).*(-1.0./2.0);
t2745 = t2248.*(t111-t181+t560-t1130+t1140+t275.*(t37-t163)+t315.*(t37-t163)+t16.*(t116+t186+t776+t7.*(t131+t14.*t91))).*(-1.0./2.0);
t2756 = -t2752;
t2757 = t1722.*(t587-t756+t1043-t1401+t1402+t893.*(t37-t163)+t895.*(t37-t163)+t16.*(t116+t186+t776+t7.*(t131+t14.*t91)).*7.35522e-1).*(-1.0./2.0);
t2760 = (t2308.*t2348)./2.0;
t2764 = (t1926.*t2554)./2.0;
t2771 = t2087.*(t688-t844+t1125-t1501+t1646+t9.*(t37-t163).*6.1597e-2+t17.*(t172-t220)).*(-1.0./2.0);
t2773 = (t2087.*(t688-t844+t1125-t1501+t1646+t9.*(t37-t163).*6.1597e-2+t17.*(t172-t220)))./2.0;
t2780 = t1823.*(t587-t756+t1043-t1401+t1402+t893.*(t37-t163)+t895.*(t37-t163)+t16.*(t116+t186+t776+t7.*(t131+t14.*t91)).*7.35522e-1).*(-1.0./2.0);
t2788 = t2133.*(t1847-t2168).*(-1.0./2.0);
t2790 = (t2133.*(t1847-t2168))./2.0;
t2793 = -t2792;
t2801 = t2448.*(t1587-t1919).*(-1.0./2.0);
t2803 = (t2448.*(t1587-t1919))./2.0;
t2806 = t2173.*(t1847-t2168).*(-1.0./2.0);
t2807 = (t2272.*t2448)./2.0;
t2811 = (t2277.*t2449)./2.0;
t2854 = t2562.*(t1582-t1924).*(-1.0./2.0);
t2855 = (t2271.*t2562)./2.0;
t2865 = t2160.*(t587-t756+t1043-t1401+t1402+t893.*(t37-t163)+t895.*(t37-t163)+t16.*(t116+t186+t776+t7.*(t131+t14.*t91)).*7.35522e-1).*(-1.0./2.0);
t2866 = (t2160.*(t587-t756+t1043-t1401+t1402+t893.*(t37-t163)+t895.*(t37-t163)+t16.*(t116+t186+t776+t7.*(t131+t14.*t91)).*7.35522e-1))./2.0;
t2867 = t2481.*(t111-t181+t560-t1130+t1140+t275.*(t37-t163)+t315.*(t37-t163)+t16.*(t116+t186+t776+t7.*(t131+t14.*t91))).*(-1.0./2.0);
t2868 = (t2481.*(t111-t181+t560-t1130+t1140+t275.*(t37-t163)+t315.*(t37-t163)+t16.*(t116+t186+t776+t7.*(t131+t14.*t91))))./2.0;
t2872 = (t2135.*t2630)./2.0;
t2875 = t2355.*(t1847-t2168).*(-1.0./2.0);
t2877 = (t2355.*(t1847-t2168))./2.0;
t2880 = -t2878;
t2883 = -t2882;
t2884 = t2359.*(t1847-t2168).*(-1.0./2.0);
t2885 = (t2359.*(t1847-t2168))./2.0;
t2905 = t2471.*(t1847-t2168).*(-1.0./2.0);
t2911 = (t1524.*t2842)./2.0;
t2916 = t1231+t1232+t1297+t1301+t1314+t1337+t1350+t1351+t1361+t1370+t1393+t1408;
t2921 = (t1662.*t2842)./2.0;
t2924 = -t2923;
t2933 = t2554.*(t688-t844+t1125-t1501+t1646+t9.*(t37-t163).*6.1597e-2+t17.*(t172-t220)).*(-1.0./2.0);
t2956 = (t1056.*t2937)./2.0;
t2962 = (t1189.*t2937)./2.0;
t2976 = (t2173.*t2842)./2.0;
t2987 = (t1723.*t2937)./2.0;
t2991 = t540+t703+t717+t829+t2345+t2715;
t2992 = t610+t723+t742+t831+t2941;
t2998 = t1327+t1328+t1369+t1413+t1415+t1421+t1476+t1486+t1544+t1545+t1703+t1710;
t2999 = (t2359.*t2842)./2.0;
t3000 = (t1879.*t2937)./2.0;
t3010 = t8.*(-t551+t723+t742+t831+t2941).*8.7635794675e-3;
t3014 = (t2937.*(t676+t692-t826+t845-t1467))./2.0;
t3015 = (t2471.*t2842)./2.0;
t3037 = t1028+t1127+t1148+t1223+t2408+t2737;
t3045 = t8.*(-t996+t1127+t1148+t1223+t2408+t2737).*5.2585e-3;
t3048 = (t1784.*(-t551+t723+t742+t831+t2941))./2.0;
t3059 = t1537.*(t111-t181-t1130+t1140+t2343+t2713+t275.*(t37-t163)+t315.*(t37-t163)).*(-1.0./2.0);
t3061 = (t1942.*(-t551+t723+t742+t831+t2941))./2.0;
t3063 = (t1265.*(-t996+t1127+t1148+t1223+t2408+t2737))./2.0;
t3072 = t1649.*(t111-t181-t1130+t1140+t2343+t2713+t275.*(t37-t163)+t315.*(t37-t163)).*(-1.0./2.0);
t3073 = t2915.*(t1847-t2168).*(-1.0./2.0);
t3074 = (t2915.*(t1847-t2168))./2.0;
t3080 = (t1618.*(-t996+t1127+t1148+t1223+t2408+t2737))./2.0;
t3084 = t2937.*(t1847-t2168).*(-1.0./2.0);
t3097 = ((t385-t428).*(t587-t756-t1401+t1402+t2398+t2739+t893.*(t37-t163)+t895.*(t37-t163)))./2.0;
t3098 = t1134.*(t587-t756-t1401+t1402+t2398+t2739+t893.*(t37-t163)+t895.*(t37-t163)).*(-1.0./2.0);
t3102 = (t2333.*(-t551+t723+t742+t831+t2941))./2.0;
t3103 = (t1977.*(-t996+t1127+t1148+t1223+t2408+t2737))./2.0;
t3105 = t2219.*(t111-t181-t1130+t1140+t2343+t2713+t275.*(t37-t163)+t315.*(t37-t163)).*(-1.0./2.0);
t3106 = t2248.*(t111-t181-t1130+t1140+t2343+t2713+t275.*(t37-t163)+t315.*(t37-t163)).*(-1.0./2.0);
t3110 = t1722.*(t587-t756-t1401+t1402+t2398+t2739+t893.*(t37-t163)+t895.*(t37-t163)).*(-1.0./2.0);
t3112 = (-t996+t1127+t1148+t1223+t2408+t2737).*(-t551-t570+t723+t742+t831+t8.*(t116+t186+t776+t7.*(t131+t14.*t91))).*(-1.0./2.0);
t3115 = ((-t996+t1127+t1148+t1223+t2408+t2737).*(-t551-t570+t723+t742+t831+t8.*(t116+t186+t776+t7.*(t131+t14.*t91))))./2.0;
t3116 = (-t551+t723+t742+t831+t2941).*(-t996-t1045+t1127+t1148+t1223+t8.*(t116+t186+t776+t7.*(t131+t14.*t91)).*1.666555).*(-1.0./2.0);
t3117 = ((-t551+t723+t742+t831+t2941).*(-t996-t1045+t1127+t1148+t1223+t8.*(t116+t186+t776+t7.*(t131+t14.*t91)).*1.666555))./2.0;
t3126 = t1823.*(t587-t756-t1401+t1402+t2398+t2739+t893.*(t37-t163)+t895.*(t37-t163)).*(-1.0./2.0);
t3133 = t2160.*(t587-t756-t1401+t1402+t2398+t2739+t893.*(t37-t163)+t895.*(t37-t163)).*(-1.0./2.0);
t3134 = (t2160.*(t587-t756-t1401+t1402+t2398+t2739+t893.*(t37-t163)+t895.*(t37-t163)))./2.0;
t3135 = t2481.*(t111-t181-t1130+t1140+t2343+t2713+t275.*(t37-t163)+t315.*(t37-t163)).*(-1.0./2.0);
t3136 = (t2481.*(t111-t181-t1130+t1140+t2343+t2713+t275.*(t37-t163)+t315.*(t37-t163)))./2.0;
t3143 = ((t587-t756-t1401+t1402+t2398+t2739+t893.*(t37-t163)+t895.*(t37-t163)).*(t111-t181+t560-t1130+t1140+t275.*(t37-t163)+t315.*(t37-t163)+t16.*(t116+t186+t776+t7.*(t131+t14.*t91))))./2.0;
t3144 = ((t587-t756+t1043-t1401+t1402+t893.*(t37-t163)+t895.*(t37-t163)+t16.*(t116+t186+t776+t7.*(t131+t14.*t91)).*7.35522e-1).*(t111-t181-t1130+t1140+t2343+t2713+t275.*(t37-t163)+t315.*(t37-t163)))./2.0;
t3151 = t698+t823+t849+t853+t1123+t2710+t2944;
t3154 = t9.*(t688-t844+t1125+t2711+t9.*(t37-t163).*6.1597e-2+t17.*(t172-t220)+t9.*(t2344-t2712)).*(-2.2652974317e-2);
t3160 = t1658.*(t688-t844+t1125+t2711+t9.*(t37-t163).*6.1597e-2+t17.*(t172-t220)+t9.*(t2344-t2712)).*(-1.0./2.0);
t3161 = (t1658.*(t688-t844+t1125+t2711+t9.*(t37-t163).*6.1597e-2+t17.*(t172-t220)+t9.*(t2344-t2712)))./2.0;
t3168 = t1096+t1227+t1230+t1238+t1389+t2735+t2950;
t3171 = t9.*(t1114-t1224+t1390+t2736+t9.*(t37-t163).*4.5305948634e-2+t17.*(t172-t220).*7.35522e-1+t9.*(t2344-t2712).*7.35522e-1).*(-3.07985e-2);
t3173 = t1184.*(t1114-t1224+t1390+t2736+t9.*(t37-t163).*4.5305948634e-2+t17.*(t172-t220).*7.35522e-1+t9.*(t2344-t2712).*7.35522e-1).*(-1.0./2.0);
t3174 = (t1184.*(t1114-t1224+t1390+t2736+t9.*(t37-t163).*4.5305948634e-2+t17.*(t172-t220).*7.35522e-1+t9.*(t2344-t2712).*7.35522e-1))./2.0;
t3176 = t2087.*(t688-t844+t1125+t2711+t9.*(t37-t163).*6.1597e-2+t17.*(t172-t220)+t9.*(t2344-t2712)).*(-1.0./2.0);
t3177 = (t2087.*(t688-t844+t1125+t2711+t9.*(t37-t163).*6.1597e-2+t17.*(t172-t220)+t9.*(t2344-t2712)))./2.0;
t3179 = t1635.*(t1114-t1224+t1390+t2736+t9.*(t37-t163).*4.5305948634e-2+t17.*(t172-t220).*7.35522e-1+t9.*(t2344-t2712).*7.35522e-1).*(-1.0./2.0);
t3181 = (t1635.*(t1114-t1224+t1390+t2736+t9.*(t37-t163).*4.5305948634e-2+t17.*(t172-t220).*7.35522e-1+t9.*(t2344-t2712).*7.35522e-1))./2.0;
t3185 = t1926.*(t1114-t1224+t1390+t2736+t9.*(t37-t163).*4.5305948634e-2+t17.*(t172-t220).*7.35522e-1+t9.*(t2344-t2712).*7.35522e-1).*(-1.0./2.0);
t3187 = (t1926.*(t1114-t1224+t1390+t2736+t9.*(t37-t163).*4.5305948634e-2+t17.*(t172-t220).*7.35522e-1+t9.*(t2344-t2712).*7.35522e-1))./2.0;
t3191 = t2307.*(t1114-t1224+t1390+t2736+t9.*(t37-t163).*4.5305948634e-2+t17.*(t172-t220).*7.35522e-1+t9.*(t2344-t2712).*7.35522e-1).*(-1.0./2.0);
t3194 = t2554.*(t688-t844+t1125+t2711+t9.*(t37-t163).*6.1597e-2+t17.*(t172-t220)+t9.*(t2344-t2712)).*(-1.0./2.0);
t3200 = ((t1114-t1224+t1390+t2736+t9.*(t37-t163).*4.5305948634e-2+t17.*(t172-t220).*7.35522e-1+t9.*(t2344-t2712).*7.35522e-1).*(t688-t844+t1125-t1501+t1646+t9.*(t37-t163).*6.1597e-2+t17.*(t172-t220)))./2.0;
t1613 = -t1609;
t1739 = -t1736;
t1834 = -t1831;
t1950 = -t1949;
t2058 = -t2056;
t2084 = -t2080;
t2113 = -t2111;
t2132 = -t2130;
t2223 = t2144.*1.225946;
t2224 = t2144.*1.666555;
t2225 = t2142.*1.225946;
t2239 = t673+t825+t860+t868+t1135+t1165;
t2243 = (t17.*t2227)./2.0;
t2247 = (t9.*t16.*t2227)./2.0;
t2251 = (t9.*t2246)./2.0;
t2256 = (t16.*t17.*t2246)./2.0;
t2257 = (t143.*t2227)./2.0;
t2260 = (t109.*t2246)./2.0;
t2263 = (t177.*t2227)./2.0;
t2266 = t2142.*5.034347249e-2;
t2269 = t2144.*1.4653732538e-2;
t2276 = -t2270;
t2296 = t2246.*(t41-t154).*(-1.0./2.0);
t2298 = -t2293;
t2312 = t2227.*(t164+t9.*(t30-t150)).*(-1.0./2.0);
t2313 = -t2310;
t2316 = (t661.*t2246)./2.0;
t2317 = t6.*t2262.*1.3727e-2;
t2324 = -t2322;
t2325 = -t2323;
t2340 = t1078.*t2227;
t2350 = -t2246.*(t666+t9.*(t37-t163));
t2351 = t2246.*(t666+t9.*(t37-t163));
t2358 = t127+t181+t638+t859+t863+t1130+t1153+t1489;
t2367 = (t1064.*t2262)./2.0;
t2383 = -t2376;
t2387 = -t2380;
t2389 = -t2381;
t2392 = -t2384;
t2393 = -t2385;
t2395 = -t2386;
t2413 = -t2411;
t2415 = t9.*t2349.*3.07985e-2;
t2438 = (t1454.*t2262)./2.0;
t2445 = -t2444;
t2447 = -t2446;
t2451 = -t2450;
t2459 = -t2458;
t2464 = -t2462;
t2465 = -t2463;
t2470 = (t1184.*t2349)./2.0;
t2482 = t1849+t2142;
t2483 = t723+t815+t831+t862+t1143+t1500+t1647;
t2484 = t716+t816+t844+t851+t1146+t1501+t1651;
t2485 = t1855+t2144;
t2496 = t8.*t2488;
t2497 = t16.*t2488;
t2506 = -t2504;
t2509 = -t2507;
t2517 = -t2515;
t2520 = -t2519;
t2544 = t2505.*(-7.35522e-1);
t2546 = t2505.*7.35522e-1;
t2553 = (t1635.*t2349)./2.0;
t2574 = t1925+t2241;
t2580 = t1932+t2238;
t2582 = t1931+t2240;
t2592 = t7.*t2488.*2.11820788799e-1;
t2597 = t2505.*(-3.127439544e-3);
t2607 = t17.*t2555.*3.07985e-2;
t2613 = -t2611;
t2621 = t15.*(t1923-t2238).*(-1.727815e-1);
t2624 = t626+t756+t1048+t1245+t1246+t1401+t1409+t1610;
t2632 = (t1186.*t2555)./2.0;
t2635 = -t2633;
t2639 = t1056.*(t1922-t2240).*(-1.0./2.0);
t2647 = t1189.*(t1922-t2240).*(-1.0./2.0);
t2652 = -t2651;
t2659 = -t2657;
t2660 = t1383.*(t1923-t2238).*(-1.0./2.0);
t2662 = (t1383.*(t1923-t2238))./2.0;
t2664 = -t2661;
t2672 = -t2671;
t2678 = t1118+t1209+t1225+t1242+t1397+t1614+t1737;
t2681 = (t1640.*t2555)./2.0;
t2682 = -t2680;
t2690 = (t1796.*t2488)./2.0;
t2694 = -t2692;
t2700 = -t2697;
t2703 = -t2702;
t2716 = t9.*(t1114-t1224+t1390-t1615+t1736+t9.*(t37-t163).*4.5305948634e-2+t17.*(t172-t220).*7.35522e-1).*(-3.07985e-2);
t2730 = t1709.*(t1923-t2238).*(-1.0./2.0);
t2733 = (t1709.*(t1923-t2238))./2.0;
t2734 = t1723.*(t1922-t2240).*(-1.0./2.0);
t2747 = t1184.*(t1114-t1224+t1390-t1615+t1736+t9.*(t37-t163).*4.5305948634e-2+t17.*(t172-t220).*7.35522e-1).*(-1.0./2.0);
t2749 = (t1184.*(t1114-t1224+t1390-t1615+t1736+t9.*(t37-t163).*4.5305948634e-2+t17.*(t172-t220).*7.35522e-1))./2.0;
t2758 = (t1910.*t2555)./2.0;
t2761 = (t2307.*t2349)./2.0;
t2762 = -t2760;
t2765 = -t2764;
t2768 = t1879.*(t1922-t2240).*(-1.0./2.0);
t2769 = (t1879.*(t1922-t2240))./2.0;
t2778 = t1964.*(t1923-t2238).*(-1.0./2.0);
t2779 = (t1964.*(t1923-t2238))./2.0;
t2786 = (t2131.*t2488)./2.0;
t2800 = (t2262.*t2449)./2.0;
t2808 = t1635.*(t1114-t1224+t1390-t1615+t1736+t9.*(t37-t163).*4.5305948634e-2+t17.*(t172-t220).*7.35522e-1).*(-1.0./2.0);
t2810 = -t2807;
t2812 = (t1635.*(t1114-t1224+t1390-t1615+t1736+t9.*(t37-t163).*4.5305948634e-2+t17.*(t172-t220).*7.35522e-1))./2.0;
t2814 = -t2811;
t2822 = (t1922-t2240).*(t676+t692-t826+t845-t1467).*(-1.0./2.0);
t2860 = t2349.*(t688-t844+t1125-t1501+t1646+t9.*(t37-t163).*6.1597e-2+t17.*(t172-t220)).*(-1.0./2.0);
t2861 = t1926.*(t1114-t1224+t1390-t1615+t1736+t9.*(t37-t163).*4.5305948634e-2+t17.*(t172-t220).*7.35522e-1).*(-1.0./2.0);
t2862 = (t2349.*(t688-t844+t1125-t1501+t1646+t9.*(t37-t163).*6.1597e-2+t17.*(t172-t220)))./2.0;
t2863 = (t1926.*(t1114-t1224+t1390-t1615+t1736+t9.*(t37-t163).*4.5305948634e-2+t17.*(t172-t220).*7.35522e-1))./2.0;
t2870 = t2488.*(t796-t908-t982+t1018+t1086-t1155+t7.*(t131+t14.*t91).*1.225946).*(-1.0./2.0);
t2873 = -t2872;
t2931 = t2307.*(t1114-t1224+t1390-t1615+t1736+t9.*(t37-t163).*4.5305948634e-2+t17.*(t172-t220).*7.35522e-1).*(-1.0./2.0);
t3001 = -t2999;
t3002 = -t3000;
t3009 = t16.*t2991.*8.7635794675e-3;
t3011 = -t3010;
t3016 = t127+t181+t859+t863+t1130+t1153+t2345+t2715;
t3029 = t2816.*(t1923-t2238).*(-1.0./2.0);
t3030 = (t2816.*(t1923-t2238))./2.0;
t3036 = t1035+t1093+t1137+t1221+t2407+t2741;
t3040 = t2842.*(t1922-t2240).*(-1.0./2.0);
t3046 = -t3045;
t3047 = (t1789.*t2991)./2.0;
t3049 = -t3048;
t3060 = (t1945.*t2991)./2.0;
t3064 = -t3063;
t3067 = t2488.*(-t908-t982+t1018+t1086-t1155+t2097+t2334.*1.225946).*(-1.0./2.0);
t3082 = t626+t756+t1245+t1246+t1401+t1409+t2406+t2742;
t3101 = (t2331.*t2991)./2.0;
t3113 = (t2442.*t2991)./2.0;
t3152 = t716+t816+t844+t851+t1146+t2714+t2943;
t3153 = t17.*(-t698+t815+t831+t862+t1143+t9.*(t97+t729+t2022+t2335)+t17.*(t2344-t2712)).*(-2.2652974317e-2);
t3159 = t1657.*(-t698+t815+t831+t862+t1143+t9.*(t97+t729+t2022+t2335)+t17.*(t2344-t2712)).*(-1.0./2.0);
t3169 = t1129+t1210+t1224+t1241+t1398+t2740+t2949;
t3170 = t17.*t3168.*3.07985e-2;
t3172 = (t1186.*t3168)./2.0;
t3175 = t2088.*(-t698+t815+t831+t862+t1143+t9.*(t97+t729+t2022+t2335)+t17.*(t2344-t2712)).*(-1.0./2.0);
t3180 = (t1640.*t3168)./2.0;
t3183 = (t1910.*t3168)./2.0;
t3184 = t2348.*(-t698+t815+t831+t862+t1143+t9.*(t97+t729+t2022+t2335)+t17.*(t2344-t2712)).*(-1.0./2.0);
t3186 = t2349.*(t688-t844+t1125+t2711+t9.*(t37-t163).*6.1597e-2+t17.*(t172-t220)+t9.*(t2344-t2712)).*(-1.0./2.0);
t3188 = (t2349.*(t688-t844+t1125+t2711+t9.*(t37-t163).*6.1597e-2+t17.*(t172-t220)+t9.*(t2344-t2712)))./2.0;
t3189 = (t2308.*t3168)./2.0;
t3190 = t2555.*(-t698+t815+t831+t862+t1143+t9.*(t97+t729+t2022+t2335)+t17.*(t2344-t2712)).*(-1.0./2.0);
t3193 = (t2555.*(-t698+t815+t831+t862+t1143+t9.*(t97+t729+t2022+t2335)+t17.*(t2344-t2712)))./2.0;
t3201 = ((t688-t844+t1125+t2711+t9.*(t37-t163).*6.1597e-2+t17.*(t172-t220)+t9.*(t2344-t2712)).*(t1114-t1224+t1390-t1615+t1736+t9.*(t37-t163).*4.5305948634e-2+t17.*(t172-t220).*7.35522e-1))./2.0;
t3214 = t1424+t1480+t1481+t1504+t1507+t1508+t1546+t1547+t2754+t2755+t2959+t2961;
t2253 = -t2251;
t2261 = -t2260;
t2275 = -t2269;
t2318 = -t2317;
t2371 = -t2367;
t2416 = -t2415;
t2439 = -t2438;
t2486 = t8.*t2482;
t2487 = t16.*t2482;
t2490 = t9.*t2485;
t2491 = t17.*t2485;
t2501 = -t2496;
t2538 = t2497.*7.35522e-1;
t2539 = t2496.*1.666555;
t2540 = t2497.*1.666555;
t2564 = t1940+t2225;
t2566 = t1947+t2223;
t2569 = t1946+t2224;
t2576 = t7.*t2482.*2.11820788799e-1;
t2577 = t17.*t2483.*2.2652974317e-2;
t2584 = t893.*t2485;
t2585 = t895.*t2485;
t2586 = t15.*t2485.*2.11820788799e-1;
t2590 = t2496.*2.3526756935e-2;
t2591 = t2497.*1.00241616695e-1;
t2610 = -t2607;
t2620 = t7.*t2574.*1.727815e-1;
t2634 = -t2632;
t2636 = (t1524.*t2485)./2.0;
t2656 = (t1379.*t2574)./2.0;
t2663 = (t1657.*t2483)./2.0;
t2669 = (t1662.*t2485)./2.0;
t2679 = t1129+t1210+t1224+t1241+t1398+t1615+t1739;
t2683 = -t2681;
t2688 = (t1796.*t2482)./2.0;
t2689 = (t1802.*t2485)./2.0;
t2717 = t17.*t2678.*3.07985e-2;
t2728 = (t1711.*t2574)./2.0;
t2746 = (t1186.*t2678)./2.0;
t2759 = -t2758;
t2763 = -t2761;
t2770 = (t2088.*t2483)./2.0;
t2776 = t2574.*(t186-t373-t503+t646+t686+t776+t7.*(t131+t14.*t91)).*(-1.0./2.0);
t2782 = (t2131.*t2482)./2.0;
t2784 = (t2133.*t2485)./2.0;
t2787 = -t2786;
t2797 = t2159+t2497;
t2798 = (t2173.*t2485)./2.0;
t2802 = -t2800;
t2809 = (t1640.*t2678)./2.0;
t2856 = (t1910.*t2678)./2.0;
t2857 = (t2348.*t2483)./2.0;
t2864 = t2482.*(t796-t908-t982+t1018+t1086-t1155+t7.*(t131+t14.*t91).*1.225946).*(-1.0./2.0);
t2869 = (t2355.*t2485)./2.0;
t2879 = (t2359.*t2485)./2.0;
t2902 = (t2471.*t2485)./2.0;
t2932 = (t2483.*t2555)./2.0;
t2934 = (t2308.*t2678)./2.0;
t3026 = (t2574.*t2815)./2.0;
t3044 = t16.*t3036.*5.2585e-3;
t3062 = (t1263.*t3036)./2.0;
t3065 = t2482.*(-t908-t982+t1018+t1086-t1155+t2097+t2334.*1.225946).*(-1.0./2.0);
t3066 = (t2485.*t2915)./2.0;
t3078 = t1424+t1480+t1481+t1504+t1507+t1508+t1546+t1547+t1718+t1719+t1832+t1834;
t3079 = (t1617.*t3036)./2.0;
t3083 = (t2485.*t2937)./2.0;
t3099 = (t1972.*t3036)./2.0;
t3104 = -t3101;
t3111 = (t2167.*t3036)./2.0;
t3192 = -t3189;
t3196 = (t2483.*t3168)./2.0;
t3198 = t2678.*(-t698+t815+t831+t862+t1143+t9.*(t97+t729+t2022+t2335)+t17.*(t2344-t2712)).*(-1.0./2.0);
t3199 = (t2678.*(-t698+t815+t831+t862+t1143+t9.*(t97+t729+t2022+t2335)+t17.*(t2344-t2712)))./2.0;
t3217 = t950+t964+t1169+t1173+t1175+t1247+t1248+t1287+t1295+t1318+t1521+t1538+t1567+t1771+t1779+t1806+t1809+t1895+t1901+t1920+t2020+t2021+t2055+t2176+t2311+t2314+t2315+t2356+t2467+t2470;
t3219 = t1057+t1060+t1108+t1149+t1167+t1451+t1464+t1482+t1532+t1534+t1652+t1656+t1773+t1778+t1782+t1791+t1801+t1808+t1824+t1861+t1888+t1890+t1907+t1944+t1961+t2170+t2183+t2184+t2190+t2194+t2321+t2480+t2493+t2500+t2513+t2552+t2553;
t2489 = -t2486;
t2498 = -t2491;
t2528 = t2487.*7.35522e-1;
t2529 = t2486.*1.666555;
t2530 = t2487.*1.666555;
t2534 = t2490.*7.35522e-1;
t2535 = t2491.*7.35522e-1;
t2542 = -t2539;
t2573 = t2486.*2.3526756935e-2;
t2575 = t2487.*1.00241616695e-1;
t2581 = -t2577;
t2587 = t2491.*(-3.127439544e-3);
t2588 = t2490.*(-7.735484874e-3);
t2594 = -t2590;
t2616 = t7.*t2564.*1.727815e-1;
t2619 = t15.*t2566.*1.727815e-1;
t2637 = (t1056.*t2569)./2.0;
t2644 = (t1189.*t2569)./2.0;
t2653 = (t1379.*t2564)./2.0;
t2654 = (t1383.*t2566)./2.0;
t2667 = -t2663;
t2691 = -t2689;
t2718 = -t2717;
t2722 = (t1711.*t2564)./2.0;
t2725 = (t1709.*t2566)./2.0;
t2729 = -t2728;
t2732 = (t1723.*t2569)./2.0;
t2748 = -t2746;
t2766 = (t1879.*t2569)./2.0;
t2772 = -t2770;
t2774 = t2564.*(t186-t373-t503+t646+t686+t776+t7.*(t131+t14.*t91)).*(-1.0./2.0);
t2775 = (t1964.*t2566)./2.0;
t2783 = -t2782;
t2785 = -t2784;
t2791 = t2150+t2487;
t2795 = -t9.*(t2486+t16.*(t1447-t1844));
t2796 = -t17.*(t2486+t16.*(t1447-t1844));
t2799 = t2161+t2501;
t2813 = -t2809;
t2817 = t9.*(t2486+t16.*(t1447-t1844)).*(-7.35522e-1);
t2818 = t17.*(t2486+t16.*(t1447-t1844)).*(-7.35522e-1);
t2819 = (t2569.*(t676+t692-t826+t845-t1467))./2.0;
t2827 = t9.*(t2486+t16.*(t1447-t1844)).*(-3.127439544e-3);
t2828 = t2233+t2538;
t2829 = t17.*(t2486+t16.*(t1447-t1844)).*(-7.735484874e-3);
t2830 = t2235+t2540;
t2831 = t8.*(t2486+t16.*(t1447-t1844)).*(-8.7635794675e-3);
t2832 = t17.*(t2486+t16.*(t1447-t1844)).*7.735484874e-3;
t2834 = t8.*(t2486+t16.*(t1447-t1844)).*8.7635794675e-3;
t2835 = t16.*t2797.*8.7635794675e-3;
t2858 = -t2856;
t2859 = -t2857;
t2871 = -t2869;
t2881 = -t2879;
t2890 = (t1537.*t2797)./2.0;
t2900 = (t1649.*t2797)./2.0;
t2903 = t1784.*(t2486+t16.*(t1447-t1844)).*(-1.0./2.0);
t2904 = (t1784.*(t2486+t16.*(t1447-t1844)))./2.0;
t2908 = (t1789.*t2797)./2.0;
t2926 = t1942.*(t2486+t16.*(t1447-t1844)).*(-1.0./2.0);
t2928 = (t1945.*t2797)./2.0;
t2955 = (t2219.*t2797)./2.0;
t2958 = (t2248.*t2797)./2.0;
t2979 = t2333.*(t2486+t16.*(t1447-t1844)).*(-1.0./2.0);
t2980 = (t2331.*t2797)./2.0;
t2989 = ((t2486+t16.*(t1447-t1844)).*(-t996-t1045+t1127+t1148+t1223+t8.*(t116+t186+t776+t7.*(t131+t14.*t91)).*1.666555))./2.0;
t2994 = (t2442.*t2797)./2.0;
t3005 = (t2481.*t2797)./2.0;
t3020 = t9.*(t2491+t9.*(t2486+t16.*(t1447-t1844))).*(-2.2652974317e-2);
t3025 = (t2564.*t2815)./2.0;
t3027 = (t2566.*t2816)./2.0;
t3038 = t2797.*(t587-t756+t1043-t1401+t1402+t893.*(t37-t163)+t895.*(t37-t163)+t16.*(t116+t186+t776+t7.*(t131+t14.*t91)).*7.35522e-1).*(-1.0./2.0);
t3039 = (t2569.*t2842)./2.0;
t3054 = t1658.*(t2491+t9.*(t2486+t16.*(t1447-t1844))).*(-1.0./2.0);
t3055 = (t1658.*(t2491+t9.*(t2486+t16.*(t1447-t1844))))./2.0;
t3070 = -t3066;
t3089 = t2087.*(t2491+t9.*(t2486+t16.*(t1447-t1844))).*(-1.0./2.0);
t3091 = (t2087.*(t2491+t9.*(t2486+t16.*(t1447-t1844))))./2.0;
t3100 = -t3099;
t3108 = t2349.*(t2491+t9.*(t2486+t16.*(t1447-t1844))).*(-1.0./2.0);
t3109 = (t2349.*(t2491+t9.*(t2486+t16.*(t1447-t1844))))./2.0;
t3129 = t2554.*(t2491+t9.*(t2486+t16.*(t1447-t1844))).*(-1.0./2.0);
t3147 = ((t2491+t9.*(t2486+t16.*(t1447-t1844))).*(t1114-t1224+t1390-t1615+t1736+t9.*(t37-t163).*4.5305948634e-2+t17.*(t172-t220).*7.35522e-1))./2.0;
t3163 = (t2486+t16.*(t1447-t1844)).*(-t996+t1127+t1148+t1223+t2408+t2737).*(-1.0./2.0);
t3165 = (t2797.*t3036)./2.0;
t3182 = t2797.*(t587-t756-t1401+t1402+t2398+t2739+t893.*(t37-t163)+t895.*(t37-t163)).*(-1.0./2.0);
t3197 = -t3196;
t3204 = t1254+t1279+t1307+t1309+t1313+t1329+t1340+t1356+t1360+t1377+t1891+t1915+t2069+t2084+t2242+t2357+t2414+t2416;
t3210 = ((t2491+t9.*(t2486+t16.*(t1447-t1844))).*(t1114-t1224+t1390+t2736+t9.*(t37-t163).*4.5305948634e-2+t17.*(t172-t220).*7.35522e-1+t9.*(t2344-t2712).*7.35522e-1))./2.0;
t3215 = t1298+t1306+t1326+t1359+t1364+t1365+t1376+t1395+t1410+t1502+t1511+t1557+t1559+t2034+t2050+t2382+t2395+t2433+t2606+t2610+t2613;
t3218 = t927+t975+t1195+t1201+t1203+t1207+t1259+t1308+t1311+t1324+t1332+t1363+t1368+t1381+t1552+t1633+t1643+t1928+t1930+t2037+t2040+t2051+t2125+t2132+t2222+t2387+t2389+t2412+t2469+t2506+t2509+t2609+t2634+t2635;
t3223 = t722+t740+t784+t1065+t1075+t1177+t1204+t1208+t1528+t1569+t1578+t1731+t1748+t1818+t1857+t1867+t1875+t1877+t1908+t1935+t1941+t2044+t2062+t2077+t2137+t2232+t2237+t2300+t2338+t2377+t2392+t2464+t2465+t2473+t2646+t2659+t2664+t2672+t2682+t2683;
t3227 = t817+t1150+t1158+t1269+t1283+t1317+t1466+t1492+t1515+t1517+t1541+t1542+t1644+t1648+t1735+t1755+t1770+t1793+t1822+t1825+t1826+t1837+t1914+t1969+t1971+t1975+t2006+t2026+t2067+t2070+t2092+t2116+t2254+t2255+t2328+t2332+t2336+t2459+t2461+t2514+t2517+t2518+t2612+t2652+t2694+t2759+t2762+t2763+t2765;
t3228 = t1382+t1396+t1405+t1426+t1478+t1493+t1512+t1613+t1623+t2243+t2253+t2436+t2437+t2753+t2756+t3072+t3098+t3153+t3154+t3170+t3171;
t3234 = t1072+t1103+t1124+t1162+t1367+t1386+t1435+t1455+t1469+t1525+t1570+t1577+t1626+t1672+t1679+t1759+t1762+t1785+t1786+t1792+t1798+t1800+t1811+t1948+t1951+t1956+t1981+t2015+t2027+t2028+t2031+t2032+t2071+t2110+t2113+t2114+t2118+t2154+t2226+t2245+t2274+t2312+t2316+t2494+t2495+t2533+t2541+t2593+t2595+t2699+t2700+t2701+t2703+t2705+t2707+t2866+t2868+t2931+t2932+t2933+t2934;
t3237 = t1341+t1342+t1347+t1371+t1385+t1404+t1411+t1417+t1423+t1499+t1510+t1641+t1726+t1741+t2047+t2048+t2188+t2193+t2247+t2249+t2256+t2425+t2429+t2911+t2956+t3009+t3011+t3044+t3046+t3059+t3097+t3159+t3161+t3172+t3174;
t3240 = t734+t749+t794+t1070+t1074+t1082+t1105+t1250+t1343+t1353+t1566+t1642+t1650+t1705+t1706+t1865+t1899+t1909+t1950+t1967+t2041+t2054+t2058+t2103+t2105+t2250+t2257+t2261+t2686+t2793+t2843+t2845+t2921+t2922+t2924+t2962+t3047+t3049+t3062+t3064+t3105+t3110+t3175+t3177+t3180+t3181;
t3241 = t885+t1171+t1239+t1322+t1333+t1366+t1523+t1551+t1555+t1619+t1752+t1760+t1761+t1767+t1769+t1839+t1873+t1876+t1905+t1927+t1929+t2016+t2045+t2076+t2081+t2083+t2115+t2258+t2263+t2296+t2368+t2511+t2512+t2558+t2648+t2649+t2673+t2789+t2917+t2919+t2938+t2939+t2976+t2987+t3060+t3061+t3079+t3080+t3106+t3126+t3183+t3184+t3187+t3188;
t2532 = -t2529;
t2537 = -t2535;
t2579 = -t2573;
t2655 = -t2654;
t2724 = -t2722;
t2726 = -t2725;
t2767 = -t2766;
t2777 = -t2775;
t2794 = t2152+t2489;
t2804 = t9.*t2799;
t2805 = t17.*t2799;
t2823 = t2228+t2528;
t2824 = t2229+t2530;
t2826 = t16.*t2791.*8.7635794675e-3;
t2833 = t2236+t2542;
t2838 = t8.*t2799.*8.7635794675e-3;
t2847 = t8.*(t2529+t16.*(t1447-t1844).*1.666555).*(-5.2585e-3);
t2848 = t8.*(t2529+t16.*(t1447-t1844).*1.666555).*5.2585e-3;
t2849 = t16.*t2830.*5.2585e-3;
t2886 = (t1537.*t2791)./2.0;
t2891 = t2828.*(t385-t428).*(-1.0./2.0);
t2892 = (t1134.*t2828)./2.0;
t2894 = t1265.*(t2529+t16.*(t1447-t1844).*1.666555).*(-1.0./2.0);
t2895 = (t1265.*(t2529+t16.*(t1447-t1844).*1.666555))./2.0;
t2896 = (t1263.*t2830)./2.0;
t2899 = (t1649.*t2791)./2.0;
t2901 = (t1789.*t2791)./2.0;
t2907 = t1618.*(t2529+t16.*(t1447-t1844).*1.666555).*(-1.0./2.0);
t2909 = (t1784.*t2799)./2.0;
t2912 = (t1617.*t2830)./2.0;
t2920 = (t1722.*t2828)./2.0;
t2925 = (t1945.*t2791)./2.0;
t2930 = (t1942.*t2799)./2.0;
t2936 = (t1823.*t2828)./2.0;
t2945 = t1977.*(t2529+t16.*(t1447-t1844).*1.666555).*(-1.0./2.0);
t2946 = (t1972.*t2830)./2.0;
t2954 = (t2219.*t2791)./2.0;
t2957 = (t2248.*t2791)./2.0;
t2969 = ((t2529+t16.*(t1447-t1844).*1.666555).*(-t551-t570+t723+t742+t831+t8.*(t116+t186+t776+t7.*(t131+t14.*t91))))./2.0;
t2971 = (t2160.*t2828)./2.0;
t2973 = (t2167.*t2830)./2.0;
t2977 = (t2331.*t2791)./2.0;
t2981 = -t2980;
t2982 = (t2333.*t2799)./2.0;
t2988 = (t2442.*t2791)./2.0;
t2990 = -t2989;
t2995 = t2799.*(-t996-t1045+t1127+t1148+t1223+t8.*(t116+t186+t776+t7.*(t131+t14.*t91)).*1.666555).*(-1.0./2.0);
t2996 = (t2799.*(-t996-t1045+t1127+t1148+t1223+t8.*(t116+t186+t776+t7.*(t131+t14.*t91)).*1.666555))./2.0;
t2997 = t2828.*(t111-t181+t560-t1130+t1140+t275.*(t37-t163)+t315.*(t37-t163)+t16.*(t116+t186+t776+t7.*(t131+t14.*t91))).*(-1.0./2.0);
t3003 = (t2481.*t2791)./2.0;
t3006 = -t3005;
t3007 = t2490+t2796;
t3008 = t2498+t2795;
t3017 = t2534+t2818;
t3028 = -t3027;
t3032 = t9.*(t2535+t9.*(t2486+t16.*(t1447-t1844)).*7.35522e-1).*(-3.07985e-2);
t3035 = t2791.*(t587-t756+t1043-t1401+t1402+t893.*(t37-t163)+t895.*(t37-t163)+t16.*(t116+t186+t776+t7.*(t131+t14.*t91)).*7.35522e-1).*(-1.0./2.0);
t3042 = t1184.*(t2535+t9.*(t2486+t16.*(t1447-t1844)).*7.35522e-1).*(-1.0./2.0);
t3043 = (t1184.*(t2535+t9.*(t2486+t16.*(t1447-t1844)).*7.35522e-1))./2.0;
t3068 = t1635.*(t2535+t9.*(t2486+t16.*(t1447-t1844)).*7.35522e-1).*(-1.0./2.0);
t3071 = (t1635.*(t2535+t9.*(t2486+t16.*(t1447-t1844)).*7.35522e-1))./2.0;
t3086 = t1926.*(t2535+t9.*(t2486+t16.*(t1447-t1844)).*7.35522e-1).*(-1.0./2.0);
t3087 = (t1926.*(t2535+t9.*(t2486+t16.*(t1447-t1844)).*7.35522e-1))./2.0;
t3121 = t2307.*(t2535+t9.*(t2486+t16.*(t1447-t1844)).*7.35522e-1).*(-1.0./2.0);
t3139 = ((t2535+t9.*(t2486+t16.*(t1447-t1844)).*7.35522e-1).*(t688-t844+t1125-t1501+t1646+t9.*(t37-t163).*6.1597e-2+t17.*(t172-t220)))./2.0;
t3156 = (t2529+t16.*(t1447-t1844).*1.666555).*(-t551+t723+t742+t831+t2941).*(-1.0./2.0);
t3157 = (t2830.*t2991)./2.0;
t3162 = (t2791.*t3036)./2.0;
t3166 = (t2799.*(-t996+t1127+t1148+t1223+t2408+t2737))./2.0;
t3167 = t2828.*(t111-t181-t1130+t1140+t2343+t2713+t275.*(t37-t163)+t315.*(t37-t163)).*(-1.0./2.0);
t3178 = t2791.*(t587-t756-t1401+t1402+t2398+t2739+t893.*(t37-t163)+t895.*(t37-t163)).*(-1.0./2.0);
t3202 = t2587+t2588+t2827+t2832;
t3206 = ((t2535+t9.*(t2486+t16.*(t1447-t1844)).*7.35522e-1).*(t688-t844+t1125+t2711+t9.*(t37-t163).*6.1597e-2+t17.*(t172-t220)+t9.*(t2344-t2712)))./2.0;
t3216 = t1378+t1380+t1382+t1396+t1405+t1426+t1478+t1493+t1512+t1613+t1623+t1716+t1717+t2243+t2253+t2563+t2581+t2583+t2675+t2716+t2718;
t3222 = t1191+t1196+t1243+t1258+t1341+t1342+t1347+t1371+t1385+t1404+t1411+t1417+t1423+t1499+t1510+t1641+t1726+t1741+t2047+t2048+t2247+t2249+t2256+t2304+t2306+t2347+t2474+t2477+t2521+t2559+t2667+t2668+t2674+t2748+t2749;
t3226 = t765+t783+t794+t1070+t1074+t1082+t1105+t1250+t1343+t1353+t1566+t1642+t1650+t1865+t1899+t1909+t1950+t1967+t2041+t2054+t2058+t2107+t2121+t2216+t2250+t2257+t2261+t2369+t2417+t2419+t2424+t2475+t2476+t2550+t2551+t2571+t2743+t2757+t2772+t2773+t2812+t2813;
t3231 = t885+t1171+t1239+t1322+t1333+t1366+t1523+t1551+t1555+t1619+t1712+t1720+t1752+t1788+t1839+t1873+t1876+t1905+t1927+t1929+t1991+t1994+t1998+t2016+t2045+t2076+t2081+t2083+t2115+t2146+t2258+t2263+t2296+t2365+t2374+t2402+t2478+t2479+t2545+t2549+t2617+t2618+t2622+t2650+t2745+t2780+t2858+t2859+t2862+t2863;
t3242 = t1072+t1103+t1124+t1162+t1367+t1386+t1435+t1455+t1469+t1525+t1626+t1695+t1759+t1762+t1772+t1792+t1800+t1811+t1948+t1951+t1956+t1981+t2027+t2028+t2071+t2113+t2118+t2128+t2154+t2212+t2226+t2245+t2274+t2302+t2305+t2312+t2316+t2400+t2420+t2423+t2561+t2641+t2642+t2676+t2677+t2841+t2853+t2952+t2953+t2964+t2965+t3001+t3002+t3100+t3102+t3103+t3104+t3134+t3136+t3191+t3192+t3193+t3194;
t3243 = t208+t790+t1252+t1427+t1453+t1518+t1527+t1632+t1758+t1787+t1859+t1860+t1955+t1958+t1959+t1978+t1979+t1993+t2108+t2134+t2145+t2155+t2169+t2215+t2313+t2340+t2351+t2379+t2404+t2460+t2466+t2536+t2614+t2684+t2687+t2727+t2731+t2851+t2887+t2983+t2984+t2985+t2986+t3014+t3015+t3111+t3113+t3115+t3117+t3143+t3144+t3197+t3199+t3200+t3201+9.213163777211224e-3;
t2820 = t2804.*7.35522e-1;
t2821 = t2805.*7.35522e-1;
t2825 = t2230+t2532;
t2836 = t2804.*3.127439544e-3;
t2837 = t2805.*7.735484874e-3;
t2840 = -t2838;
t2846 = t16.*t2824.*5.2585e-3;
t2850 = t8.*t2833.*5.2585e-3;
t2888 = t2823.*(t385-t428).*(-1.0./2.0);
t2889 = (t1134.*t2823)./2.0;
t2893 = (t1263.*t2824)./2.0;
t2897 = (t1265.*t2833)./2.0;
t2906 = (t1617.*t2824)./2.0;
t2910 = -t2909;
t2913 = (t1618.*t2833)./2.0;
t2918 = (t1722.*t2823)./2.0;
t2935 = (t1823.*t2823)./2.0;
t2940 = (t1972.*t2824)./2.0;
t2947 = -t2946;
t2948 = (t1977.*t2833)./2.0;
t2966 = (t2160.*t2823)./2.0;
t2968 = (t2167.*t2824)./2.0;
t2970 = -t2969;
t2972 = -t2971;
t2974 = t2833.*(-t551-t570+t723+t742+t831+t8.*(t116+t186+t776+t7.*(t131+t14.*t91))).*(-1.0./2.0);
t2975 = (t2833.*(-t551-t570+t723+t742+t831+t8.*(t116+t186+t776+t7.*(t131+t14.*t91))))./2.0;
t2978 = -t2977;
t2993 = t2823.*(t111-t181+t560-t1130+t1140+t275.*(t37-t163)+t315.*(t37-t163)+t16.*(t116+t186+t776+t7.*(t131+t14.*t91))).*(-1.0./2.0);
t3004 = -t3003;
t3012 = t2502+t2805;
t3013 = t2505+t2804;
t3018 = t2537+t2817;
t3019 = t17.*t3007.*2.2652974317e-2;
t3031 = t17.*t3017.*3.07985e-2;
t3041 = (t1186.*t3017)./2.0;
t3053 = (t1657.*t3007)./2.0;
t3069 = (t1640.*t3017)./2.0;
t3085 = (t1910.*t3017)./2.0;
t3088 = (t2088.*t3007)./2.0;
t3107 = (t2348.*t3007)./2.0;
t3120 = (t2308.*t3017)./2.0;
t3127 = (t2555.*t3007)./2.0;
t3137 = (t2483.*t3017)./2.0;
t3145 = (t2678.*t3007)./2.0;
t3155 = (t2824.*t2991)./2.0;
t3158 = (t2833.*(-t551+t723+t742+t831+t2941))./2.0;
t3164 = t2823.*(t111-t181-t1130+t1140+t2343+t2713+t275.*(t37-t163)+t315.*(t37-t163)).*(-1.0./2.0);
t3205 = t3017.*(-t698+t815+t831+t862+t1143+t9.*(t97+t729+t2022+t2335)+t17.*(t2344-t2712)).*(-1.0./2.0);
t3209 = (t3007.*t3168)./2.0;
t2839 = -t2837;
t2852 = -t2850;
t2898 = -t2897;
t2942 = -t2940;
t2967 = -t2966;
t3021 = t2543+t2821;
t3022 = t2546+t2820;
t3023 = t17.*t3012.*2.2652974317e-2;
t3024 = t9.*t3013.*2.2652974317e-2;
t3056 = (t1657.*t3012)./2.0;
t3057 = (t1658.*t3013)./2.0;
t3094 = (t2088.*t3012)./2.0;
t3095 = (t2087.*t3013)./2.0;
t3114 = (t2348.*t3012)./2.0;
t3118 = (t2349.*t3013)./2.0;
t3122 = -t3120;
t3128 = -t3127;
t3130 = (t2555.*t3012)./2.0;
t3132 = (t2554.*t3013)./2.0;
t3138 = -t3137;
t3146 = -t3145;
t3148 = (t2678.*t3012)./2.0;
t3150 = t3013.*(t1114-t1224+t1390-t1615+t1736+t9.*(t37-t163).*4.5305948634e-2+t17.*(t172-t220).*7.35522e-1).*(-1.0./2.0);
t3211 = (t3012.*t3168)./2.0;
t3212 = t3013.*(t1114-t1224+t1390+t2736+t9.*(t37-t163).*4.5305948634e-2+t17.*(t172-t220).*7.35522e-1+t9.*(t2344-t2712).*7.35522e-1).*(-1.0./2.0);
t3220 = t2280+t2282+t2575+t2579+t2889+t2899+t3019+t3020+t3031+t3032;
t3224 = t1999+t2004+t2266+t2275+t2636+t2637+t2826+t2834+t2846+t2848+t2886+t2888+t3041+t3043+t3053+t3055;
t3229 = t1624+t1625+t1957+t1962+t2397+t2428+t2576+t2586+t2616+t2619+t2644+t2669+t2893+t2895+t2901+t2904+t2918+t2954+t3069+t3071+t3088+t3091;
t3232 = t1687+t1690+t1691+t1694+t2082+t2162+t2276+t2285+t2318+t2320+t2373+t2388+t2653+t2655+t2688+t2691+t2732+t2798+t2906+t2907+t2925+t2926+t2935+t2957+t3085+t3087+t3107+t3109;
t3244 = t2057+t2059+t2060+t2123+t2126+t2141+t2143+t2165+t2181+t2196+t2281+t2284+t2570+t2572+t2604+t2627+t2628+t2723+t2802+t2803+t2854+t2873+t2876+t2927+t3025+t3028+t3039+t3065+t3070+t3083+t3155+t3156+t3162+t3163+t3164+t3178+t3205+t3206+t3209+t3210;
t3033 = t17.*t3021.*3.07985e-2;
t3034 = t9.*t3022.*3.07985e-2;
t3050 = (t1186.*t3021)./2.0;
t3051 = (t1184.*t3022)./2.0;
t3058 = -t3057;
t3075 = (t1635.*t3022)./2.0;
t3076 = (t1640.*t3021)./2.0;
t3090 = (t1910.*t3021)./2.0;
t3092 = (t1926.*t3022)./2.0;
t3096 = -t3095;
t3119 = -t3118;
t3123 = (t2308.*t3021)./2.0;
t3124 = (t2307.*t3022)./2.0;
t3131 = -t3130;
t3140 = (t2483.*t3021)./2.0;
t3142 = t3022.*(t688-t844+t1125-t1501+t1646+t9.*(t37-t163).*6.1597e-2+t17.*(t172-t220)).*(-1.0./2.0);
t3149 = -t3148;
t3203 = t2602+t2603+t2836+t2839;
t3207 = t3021.*(-t698+t815+t831+t862+t1143+t9.*(t97+t729+t2022+t2335)+t17.*(t2344-t2712)).*(-1.0./2.0);
t3208 = t3022.*(t688-t844+t1125+t2711+t9.*(t37-t163).*6.1597e-2+t17.*(t172-t220)+t9.*(t2344-t2712)).*(-1.0./2.0);
t3235 = t1620+t1693+t1803+t1872+t2005+t2009+t2090+t2091+t2109+t2185+t2371+t2372+t2451+t2453+t2508+t2640+t2724+t2726+t2767+t2783+t2785+t2881+t2942+t2945+t2967+t2978+t2979+t3004+t3121+t3122+t3128+t3129;
t3238 = t1217+t1256+t1443+t1472+t1699+t1700+t1813+t1828+t1838+t1880+t2199+t2203+t2206+t2210+t2221+t2410+t2439+t2441+t2520+t2523+t2548+t2658+t2774+t2777+t2819+t2864+t2871+t2902+t2968+t2970+t2988+t2990+t2993+t3035+t3138+t3139+t3146+t3147;
t3052 = -t3051;
t3077 = -t3075;
t3093 = -t3092;
t3125 = -t3123;
t3141 = -t3140;
t3221 = t2288+t2289+t2591+t2594+t2892+t2900+t3023+t3024+t3033+t3034;
t3245 = t2053+t2065+t2066+t2120+t2129+t2157+t2158+t2174+t2178+t2202+t2273+t2295+t2567+t2578+t2600+t2625+t2629+t2720+t2810+t2814+t2855+t2880+t2883+t2929+t3026+t3030+t3040+t3067+t3074+t3084+t3157+t3158+t3165+t3166+t3167+t3182+t3207+t3208+t3211+t3212;
t3225 = t1992+t1997+t2292+t2298+t2638+t2639+t2835+t2840+t2849+t2852+t2890+t2891+t3050+t3052+t3056+t3058;
t3230 = t1629+t1630+t1963+t1968+t2413+t2431+t2592+t2599+t2620+t2621+t2647+t2670+t2896+t2898+t2908+t2910+t2920+t2955+t3076+t3077+t3094+t3096;
t3233 = t1683+t1684+t1701+t1702+t2079+t2153+t2291+t2299+t2324+t2325+t2378+t2409+t2656+t2662+t2690+t2695+t2734+t2806+t2912+t2913+t2928+t2930+t2936+t2958+t3090+t3093+t3114+t3119;
t3236 = t1621+t1696+t1814+t1881+t2003+t2011+t2086+t2093+t2106+t2179+t2383+t2393+t2455+t2457+t2510+t2643+t2729+t2733+t2769+t2787+t2790+t2885+t2947+t2948+t2972+t2981+t2982+t3006+t3124+t3125+t3131+t3132;
t3239 = t1233+t1257+t1445+t1479+t1713+t1714+t1817+t1819+t1835+t1884+t2198+t2204+t2207+t2209+t2217+t2396+t2445+t2447+t2526+t2527+t2557+t2665+t2776+t2779+t2822+t2870+t2877+t2905+t2973+t2975+t2994+t2996+t2997+t3038+t3141+t3142+t3149+t3150;
M = reshape([1.6062132e+1,0.0,t3244,t3238,t3235,t3232,t3229,t3224,t3220,t3202,0.0,1.6062132e+1,t3245,t3239,t3236,t3233,t3230,t3225,t3221,t3203,t3244,t3245,t208+t790+t1252+t1427+t1453+t1632+t1758+t1787+t1959+t1978+t1979+t2108+t2155+t2169+t2313+t2340+t2351+(t688-t844+t1125+t2711+t9.*(t37-t163).*6.1597e-2+t17.*(t172-t220)+t9.*(t2344-t2712)).*(t1114-t1224+t1390+t2736+t9.*(t37-t163).*4.5305948634e-2+t17.*(t172-t220).*7.35522e-1+t9.*(t2344-t2712).*7.35522e-1)+t1568.*t1830+t1685.*t1853+t1688.*t1854+t1663.*t1886+t1721.*t2010+t1794.*t2014+t2149.*t2353+t2182.*t2499+t2448.*t2631+t2449.*t2630+t2562.*t2744+t2816.*t2915+t2842.*t2937+t2991.*t3036-t3168.*(-t698+t815+t831+t862+t1143+t9.*(t97+t729+t2022+t2335)+t17.*(t2344-t2712))+(-t1107+t1550+t1573).*(-t872+t1017+t1573.*3.228604+t1654)-t2815.*(-t908-t982+t1018+t1086-t1155+t2097+t2334.*1.225946)+(-t551+t723+t742+t831+t2941).*(-t996+t1127+t1148+t1223+t2408+t2737)+(t111-t181-t1130+t1140+t2343+t2713+t275.*(t37-t163)+t315.*(t37-t163)).*(t587-t756-t1401+t1402+t2398+t2739+t893.*(t37-t163)+t895.*(t37-t163))+9.117e-3,t3243,t3242,t3241,t3240,t3237,t3228,t3214,t3238,t3239,t3243,t18.*7.902217263149999e-6+t19.*7.902217263149999e-6+t208+t790+t1252+t1427+t1453+t1632+t1758+t1787+t1959+t1978+t1979+t2108+t2155+t2169+t2313+t2340+t2351+(t186-t373-t503+t646+t686+t776+t7.*(t131+t14.*t91)).*(t796-t908-t982+t1018+t1086-t1155+t7.*(t131+t14.*t91).*1.225946)+t2471.*(t676+t692-t826+t845-t1467)+t721.*t1403+t1079.*t1531+t1091.*t1533+t1107.*t1536+t1185.*t1897+t1454.*t1906+t1465.*t1911+t1799.*t2259+t1964.*t2355+t2167.*t2442+t2483.*t2678+(t1114-t1224+t1390-t1615+t1736+t9.*(t37-t163).*4.5305948634e-2+t17.*(t172-t220).*7.35522e-1).*(t688-t844+t1125-t1501+t1646+t9.*(t37-t163).*6.1597e-2+t17.*(t172-t220))+(t587-t756+t1043-t1401+t1402+t893.*(t37-t163)+t895.*(t37-t163)+t16.*(t116+t186+t776+t7.*(t131+t14.*t91)).*7.35522e-1).*(t111-t181+t560-t1130+t1140+t275.*(t37-t163)+t315.*(t37-t163)+t16.*(t116+t186+t776+t7.*(t131+t14.*t91)))+(-t996-t1045+t1127+t1148+t1223+t8.*(t116+t186+t776+t7.*(t131+t14.*t91)).*1.666555).*(-t551-t570+t723+t742+t831+t8.*(t116+t186+t776+t7.*(t131+t14.*t91)))+9.213163777211224e-3,t3234,t3231,t3226,t3222,t3216,t3078,t3235,t3236,t3242,t3234,(t164+t9.*(t30-t150)).*(t566+t678+t701-t745+t9.*(t30-t150).*1.2516e-2+t271.*(t30-t150))-t13.*t1027+t5.*t1068+t5.*t1425+t107.*t1730-t141.*t1724+t141.*t1892+t176.*t1900+t582.*t1513+t176.*t2029+t1059.*t1520+t661.*t2033+t1063.*t1727+t1064.*t1728+t1709.*t2133+t1711.*t2131+t1725.*t2211+t1879.*t2359+t1972.*t2331+t1977.*t2333+t2160.*t2481+t2307.*t2554+t2308.*t2555+t1898.*(t30-t150)+t5.^2.*2.009781840171224e-1+t13.^2.*2.009781840171224e-1+t13.*t14.*t1218+t6.*t13.*t1431+t13.*t14.*t1742+2.653499190169021e-2,t3227,t3223,t3218,t3215,t2998,t3232,t3233,t3241,t3231,t3227,t6.*t730+t14.*t1055-t6.*t1438+t221.*t1483+t108.*t1757+t142.*t1751+t142.*t1887+t177.*t1883+t1109.*t1535+t1379.*t1796+t1383.*t1802+t1618.*t1942+t1617.*t1945+t1723.*t2173+t1823.*t2248+t1910.*t2348+t1926.*t2349-t1894.*(t41-t154)+t6.^2.*2.70427581138582e-3+t14.^2.*2.70427581138582e-3+t14.*t15.*t1419+t7.*t14.*t1429-t14.*t15.*t1746+1.824920229252011e-2,t3219,t3217,t3204,t2916,t3229,t3230,t3240,t3226,t3223,t3219,t7.*t1034-t15.*t1054+t7.*t1434+t109.*t1743-t143.*t1729+t1119.*t1636+t1189.*t1662+t1265.*t1784+t1263.*t1789+t1635.*t2087+t1640.*t2088+t1722.*t2219+t7.^2.*1.463948544794977e-1+t15.^2.*1.463948544794977e-1+t8.*t15.*t1440+t15.*t16.*t1441+t15.*t16.*t1738+7.75868983449435e-2,t3213,t3195,t2781,t3224,t3225,t3237,t3222,t3218,t3217,t3213,t8.*t1071+t16.*t1076+t8.*t1432+t1056.*t1524+t1184.*t1658+t1186.*t1657-t1537.*(t385-t428)+t8.^2.*1.84333130519395e-4+t16.^2.*1.84333130519395e-4+t9.*t16.*t1418+t16.*t17.*t1439+1.086951076282856e-2,t3081,t2309,t3220,t3221,t3228,t3216,t3215,t3204,t3195,t3081,-t17.*t1052+t1134.*t1649-t9.*(t271-t298)+t9.^2.*2.790710518008498e-3+t17.^2.*2.790710518008498e-3+1.179456023023895e-2,t1734,t3202,t3203,t3214,t3078,t2998,t2916,t2781,t2309,t1734,4.909651967360946e-3],[10,10]);
